simulink model "model"  (R2014a)
(part 2 of 2)

  bus129 : powerlib/Measurements/Load Flow Bus  LConnTagsString=a  ID=bus129  Vbase=110000  Vref=1  Vangle=0  VLF=1  angleLF=0
      settings: AttributesFormatString=|
      | %<ID>
      | %<Vbase>V
      | %<VLF>pu
      | %<angleLF>deg.
      | %<Name>
  bus13 : powerlib/Measurements/Load Flow Bus  LConnTagsString=a  ID=bus13  Vbase=110000  Vref=1  Vangle=0  VLF=1  angleLF=0
      settings: AttributesFormatString=|
      | %<ID>
      | %<Vbase>V
      | %<VLF>pu
      | %<angleLF>deg.
      | %<Name>
  bus130 : powerlib/Measurements/Load Flow Bus  LConnTagsString=a  ID=bus130  Vbase=110000  Vref=1  Vangle=0  VLF=1  angleLF=0
      settings: AttributesFormatString=|
      | %<ID>
      | %<Vbase>V
      | %<VLF>pu
      | %<angleLF>deg.
      | %<Name>
  bus131 : powerlib/Measurements/Load Flow Bus  LConnTagsString=a  ID=bus131  Vbase=110000  Vref=1  Vangle=0  VLF=1  angleLF=0
      settings: AttributesFormatString=|
      | %<ID>
      | %<Vbase>V
      | %<VLF>pu
      | %<angleLF>deg.
      | %<Name>
  bus132 : powerlib/Measurements/Load Flow Bus  LConnTagsString=a  ID=bus132  Vbase=110000  Vref=1  Vangle=0  VLF=1  angleLF=0
      settings: AttributesFormatString=|
      | %<ID>
      | %<Vbase>V
      | %<VLF>pu
      | %<angleLF>deg.
      | %<Name>
  bus133 : powerlib/Measurements/Load Flow Bus  LConnTagsString=a  ID=bus133  Vbase=110000  Vref=1  Vangle=0  VLF=1  angleLF=0
      settings: AttributesFormatString=|
      | %<ID>
      | %<Vbase>V
      | %<VLF>pu
      | %<angleLF>deg.
      | %<Name>
  bus134 : powerlib/Measurements/Load Flow Bus  LConnTagsString=a  ID=bus134  Vbase=110000  Vref=1  Vangle=0  VLF=1  angleLF=0
      settings: AttributesFormatString=|
      | %<ID>
      | %<Vbase>V
      | %<VLF>pu
      | %<angleLF>deg.
      | %<Name>
  bus135 : powerlib/Measurements/Load Flow Bus  LConnTagsString=a  ID=bus135  Vbase=110000  Vref=1  Vangle=0  VLF=1  angleLF=0
      settings: AttributesFormatString=|
      | %<ID>
      | %<Vbase>V
      | %<VLF>pu
      | %<angleLF>deg.
      | %<Name>
  bus136 : powerlib/Measurements/Load Flow Bus  LConnTagsString=a  ID=bus136  Vbase=110000  Vref=1  Vangle=0  VLF=1  angleLF=0
      settings: AttributesFormatString=|
      | %<ID>
      | %<Vbase>V
      | %<VLF>pu
      | %<angleLF>deg.
      | %<Name>
  bus137 : powerlib/Measurements/Load Flow Bus  LConnTagsString=a  ID=bus137  Vbase=110000  Vref=1  Vangle=0  VLF=1  angleLF=0
      settings: AttributesFormatString=|
      | %<ID>
      | %<Vbase>V
      | %<VLF>pu
      | %<angleLF>deg.
      | %<Name>
  bus138 : powerlib/Measurements/Load Flow Bus  LConnTagsString=a  ID=bus138  Vbase=110000  Vref=1  Vangle=0  VLF=1  angleLF=0
      settings: AttributesFormatString=|
      | %<ID>
      | %<Vbase>V
      | %<VLF>pu
      | %<angleLF>deg.
      | %<Name>
  bus139 : powerlib/Measurements/Load Flow Bus  LConnTagsString=a  ID=bus139  Vbase=110000  Vref=1  Vangle=0  VLF=1  angleLF=0
      settings: AttributesFormatString=|
      | %<ID>
      | %<Vbase>V
      | %<VLF>pu
      | %<angleLF>deg.
      | %<Name>
  bus14 : powerlib/Measurements/Load Flow Bus  LConnTagsString=a  ID=bus14  Vbase=110000  Vref=1  Vangle=0  VLF=1  angleLF=0
      settings: AttributesFormatString=|
      | %<ID>
      | %<Vbase>V
      | %<VLF>pu
      | %<angleLF>deg.
      | %<Name>
  bus140 : powerlib/Measurements/Load Flow Bus  LConnTagsString=a  ID=bus140  Vbase=110000  Vref=1  Vangle=0  VLF=1  angleLF=0
      settings: AttributesFormatString=|
      | %<ID>
      | %<Vbase>V
      | %<VLF>pu
      | %<angleLF>deg.
      | %<Name>
  bus141 : powerlib/Measurements/Load Flow Bus  LConnTagsString=a  ID=bus141  Vbase=110000  Vref=1  Vangle=0  VLF=1  angleLF=0
      settings: AttributesFormatString=|
      | %<ID>
      | %<Vbase>V
      | %<VLF>pu
      | %<angleLF>deg.
      | %<Name>
  bus142 : powerlib/Measurements/Load Flow Bus  LConnTagsString=a  ID=bus142  Vbase=110000  Vref=1  Vangle=0  VLF=1  angleLF=0
      settings: AttributesFormatString=|
      | %<ID>
      | %<Vbase>V
      | %<VLF>pu
      | %<angleLF>deg.
      | %<Name>
  bus143 : powerlib/Measurements/Load Flow Bus  LConnTagsString=a  ID=bus143  Vbase=110000  Vref=1  Vangle=0  VLF=1  angleLF=0
      settings: AttributesFormatString=|
      | %<ID>
      | %<Vbase>V
      | %<VLF>pu
      | %<angleLF>deg.
      | %<Name>
  bus144 : powerlib/Measurements/Load Flow Bus  LConnTagsString=a  ID=bus144  Vbase=110000  Vref=1  Vangle=0  VLF=1  angleLF=0
      settings: AttributesFormatString=|
      | %<ID>
      | %<Vbase>V
      | %<VLF>pu
      | %<angleLF>deg.
      | %<Name>
  bus145 : powerlib/Measurements/Load Flow Bus  LConnTagsString=a  ID=bus145  Vbase=110000  Vref=1  Vangle=0  VLF=1  angleLF=0
      settings: AttributesFormatString=|
      | %<ID>
      | %<Vbase>V
      | %<VLF>pu
      | %<angleLF>deg.
      | %<Name>
  bus146 : powerlib/Measurements/Load Flow Bus  LConnTagsString=a  ID=bus146  Vbase=110000  Vref=1  Vangle=0  VLF=1  angleLF=0
      settings: AttributesFormatString=|
      | %<ID>
      | %<Vbase>V
      | %<VLF>pu
      | %<angleLF>deg.
      | %<Name>
  bus147 : powerlib/Measurements/Load Flow Bus  LConnTagsString=a  ID=bus147  Vbase=110000  Vref=1  Vangle=0  VLF=1  angleLF=0
      settings: AttributesFormatString=|
      | %<ID>
      | %<Vbase>V
      | %<VLF>pu
      | %<angleLF>deg.
      | %<Name>
  bus148 : powerlib/Measurements/Load Flow Bus  LConnTagsString=a  ID=bus148  Vbase=110000  Vref=1  Vangle=0  VLF=1  angleLF=0
      settings: AttributesFormatString=|
      | %<ID>
      | %<Vbase>V
      | %<VLF>pu
      | %<angleLF>deg.
      | %<Name>
  bus149 : powerlib/Measurements/Load Flow Bus  LConnTagsString=a  ID=bus149  Vbase=110000  Vref=1  Vangle=0  VLF=1  angleLF=0
      settings: AttributesFormatString=|
      | %<ID>
      | %<Vbase>V
      | %<VLF>pu
      | %<angleLF>deg.
      | %<Name>
  bus15 : powerlib/Measurements/Load Flow Bus  LConnTagsString=a  ID=bus15  Vbase=110000  Vref=1  Vangle=0  VLF=1  angleLF=0
      settings: AttributesFormatString=|
      | %<ID>
      | %<Vbase>V
      | %<VLF>pu
      | %<angleLF>deg.
      | %<Name>
  bus150 : powerlib/Measurements/Load Flow Bus  LConnTagsString=a  ID=bus150  Vbase=110000  Vref=1  Vangle=0  VLF=1  angleLF=0
      settings: AttributesFormatString=|
      | %<ID>
      | %<Vbase>V
      | %<VLF>pu
      | %<angleLF>deg.
      | %<Name>
  bus151 : powerlib/Measurements/Load Flow Bus  LConnTagsString=a  ID=bus151  Vbase=110000  Vref=1  Vangle=0  VLF=1  angleLF=0
      settings: AttributesFormatString=|
      | %<ID>
      | %<Vbase>V
      | %<VLF>pu
      | %<angleLF>deg.
      | %<Name>
  bus152 : powerlib/Measurements/Load Flow Bus  LConnTagsString=a  ID=bus152  Vbase=110000  Vref=1  Vangle=0  VLF=1  angleLF=0
      settings: AttributesFormatString=|
      | %<ID>
      | %<Vbase>V
      | %<VLF>pu
      | %<angleLF>deg.
      | %<Name>
  bus153 : powerlib/Measurements/Load Flow Bus  LConnTagsString=a  ID=bus153  Vbase=110000  Vref=1  Vangle=0  VLF=1  angleLF=0
      settings: AttributesFormatString=|
      | %<ID>
      | %<Vbase>V
      | %<VLF>pu
      | %<angleLF>deg.
      | %<Name>
  bus154 : powerlib/Measurements/Load Flow Bus  LConnTagsString=a  ID=bus154  Vbase=110000  Vref=1  Vangle=0  VLF=1  angleLF=0
      settings: AttributesFormatString=|
      | %<ID>
      | %<Vbase>V
      | %<VLF>pu
      | %<angleLF>deg.
      | %<Name>
  bus155 : powerlib/Measurements/Load Flow Bus  LConnTagsString=a  ID=bus155  Vbase=110000  Vref=1  Vangle=0  VLF=1  angleLF=0
      settings: AttributesFormatString=|
      | %<ID>
      | %<Vbase>V
      | %<VLF>pu
      | %<angleLF>deg.
      | %<Name>
  bus156 : powerlib/Measurements/Load Flow Bus  LConnTagsString=a  ID=bus156  Vbase=110000  Vref=1  Vangle=0  VLF=1  angleLF=0
      settings: AttributesFormatString=|
      | %<ID>
      | %<Vbase>V
      | %<VLF>pu
      | %<angleLF>deg.
      | %<Name>
  bus157 : powerlib/Measurements/Load Flow Bus  LConnTagsString=a  ID=bus157  Vbase=110000  Vref=1  Vangle=0  VLF=1  angleLF=0
      settings: AttributesFormatString=|
      | %<ID>
      | %<Vbase>V
      | %<VLF>pu
      | %<angleLF>deg.
      | %<Name>
  bus158 : powerlib/Measurements/Load Flow Bus  LConnTagsString=a  ID=bus158  Vbase=110000  Vref=1  Vangle=0  VLF=1  angleLF=0
      settings: AttributesFormatString=|
      | %<ID>
      | %<Vbase>V
      | %<VLF>pu
      | %<angleLF>deg.
      | %<Name>
  bus159 : powerlib/Measurements/Load Flow Bus  LConnTagsString=a  ID=bus159  Vbase=110000  Vref=1  Vangle=0  VLF=1  angleLF=0
      settings: AttributesFormatString=|
      | %<ID>
      | %<Vbase>V
      | %<VLF>pu
      | %<angleLF>deg.
      | %<Name>
  bus16 : powerlib/Measurements/Load Flow Bus  LConnTagsString=a  ID=bus16  Vbase=110000  Vref=1  Vangle=0  VLF=1  angleLF=0
      settings: AttributesFormatString=|
      | %<ID>
      | %<Vbase>V
      | %<VLF>pu
      | %<angleLF>deg.
      | %<Name>
  bus160 : powerlib/Measurements/Load Flow Bus  LConnTagsString=a  ID=bus160  Vbase=110000  Vref=1  Vangle=0  VLF=1  angleLF=0
      settings: AttributesFormatString=|
      | %<ID>
      | %<Vbase>V
      | %<VLF>pu
      | %<angleLF>deg.
      | %<Name>
  bus161 : powerlib/Measurements/Load Flow Bus  LConnTagsString=a  ID=bus161  Vbase=110000  Vref=1  Vangle=0  VLF=1  angleLF=0
      settings: AttributesFormatString=|
      | %<ID>
      | %<Vbase>V
      | %<VLF>pu
      | %<angleLF>deg.
      | %<Name>
  bus162 : powerlib/Measurements/Load Flow Bus  LConnTagsString=a  ID=bus162  Vbase=110000  Vref=1  Vangle=0  VLF=1  angleLF=0
      settings: AttributesFormatString=|
      | %<ID>
      | %<Vbase>V
      | %<VLF>pu
      | %<angleLF>deg.
      | %<Name>
  bus163 : powerlib/Measurements/Load Flow Bus  LConnTagsString=a  ID=bus163  Vbase=110000  Vref=1  Vangle=0  VLF=1  angleLF=0
      settings: AttributesFormatString=|
      | %<ID>
      | %<Vbase>V
      | %<VLF>pu
      | %<angleLF>deg.
      | %<Name>
  bus164 : powerlib/Measurements/Load Flow Bus  LConnTagsString=a  ID=bus164  Vbase=110000  Vref=1  Vangle=0  VLF=1  angleLF=0
      settings: AttributesFormatString=|
      | %<ID>
      | %<Vbase>V
      | %<VLF>pu
      | %<angleLF>deg.
      | %<Name>
  bus165 : powerlib/Measurements/Load Flow Bus  LConnTagsString=a  ID=bus165  Vbase=110000  Vref=1  Vangle=0  VLF=1  angleLF=0
      settings: AttributesFormatString=|
      | %<ID>
      | %<Vbase>V
      | %<VLF>pu
      | %<angleLF>deg.
      | %<Name>
  bus166 : powerlib/Measurements/Load Flow Bus  LConnTagsString=a  ID=bus166  Vbase=110000  Vref=1  Vangle=0  VLF=1  angleLF=0
      settings: AttributesFormatString=|
      | %<ID>
      | %<Vbase>V
      | %<VLF>pu
      | %<angleLF>deg.
      | %<Name>
  bus167 : powerlib/Measurements/Load Flow Bus  LConnTagsString=a  ID=bus167  Vbase=110000  Vref=1  Vangle=0  VLF=1  angleLF=0
      settings: AttributesFormatString=|
      | %<ID>
      | %<Vbase>V
      | %<VLF>pu
      | %<angleLF>deg.
      | %<Name>
  bus168 : powerlib/Measurements/Load Flow Bus  LConnTagsString=a  ID=bus168  Vbase=110000  Vref=1  Vangle=0  VLF=1  angleLF=0
      settings: AttributesFormatString=|
      | %<ID>
      | %<Vbase>V
      | %<VLF>pu
      | %<angleLF>deg.
      | %<Name>
  bus169 : powerlib/Measurements/Load Flow Bus  LConnTagsString=a  ID=bus169  Vbase=110000  Vref=1  Vangle=0  VLF=1  angleLF=0
      settings: AttributesFormatString=|
      | %<ID>
      | %<Vbase>V
      | %<VLF>pu
      | %<angleLF>deg.
      | %<Name>
  bus17 : powerlib/Measurements/Load Flow Bus  LConnTagsString=a  ID=bus17  Vbase=110000  Vref=1  Vangle=0  VLF=1  angleLF=0
      settings: AttributesFormatString=|
      | %<ID>
      | %<Vbase>V
      | %<VLF>pu
      | %<angleLF>deg.
      | %<Name>
  bus170 : powerlib/Measurements/Load Flow Bus  LConnTagsString=a  ID=bus170  Vbase=110000  Vref=1  Vangle=0  VLF=1  angleLF=0
      settings: AttributesFormatString=|
      | %<ID>
      | %<Vbase>V
      | %<VLF>pu
      | %<angleLF>deg.
      | %<Name>
  bus171 : powerlib/Measurements/Load Flow Bus  LConnTagsString=a  ID=bus171  Vbase=110000  Vref=1  Vangle=0  VLF=1  angleLF=0
      settings: AttributesFormatString=|
      | %<ID>
      | %<Vbase>V
      | %<VLF>pu
      | %<angleLF>deg.
      | %<Name>
  bus172 : powerlib/Measurements/Load Flow Bus  LConnTagsString=a  ID=bus172  Vbase=110000  Vref=1  Vangle=0  VLF=1  angleLF=0
      settings: AttributesFormatString=|
      | %<ID>
      | %<Vbase>V
      | %<VLF>pu
      | %<angleLF>deg.
      | %<Name>
  bus173 : powerlib/Measurements/Load Flow Bus  LConnTagsString=a  ID=bus173  Vbase=110000  Vref=1  Vangle=0  VLF=1  angleLF=0
      settings: AttributesFormatString=|
      | %<ID>
      | %<Vbase>V
      | %<VLF>pu
      | %<angleLF>deg.
      | %<Name>
  bus174 : powerlib/Measurements/Load Flow Bus  LConnTagsString=a  ID=bus174  Vbase=110000  Vref=1  Vangle=0  VLF=1  angleLF=0
      settings: AttributesFormatString=|
      | %<ID>
      | %<Vbase>V
      | %<VLF>pu
      | %<angleLF>deg.
      | %<Name>
  bus175 : powerlib/Measurements/Load Flow Bus  LConnTagsString=a  ID=bus175  Vbase=110000  Vref=1  Vangle=0  VLF=1  angleLF=0
      settings: AttributesFormatString=|
      | %<ID>
      | %<Vbase>V
      | %<VLF>pu
      | %<angleLF>deg.
      | %<Name>
  bus176 : powerlib/Measurements/Load Flow Bus  LConnTagsString=a  ID=bus176  Vbase=110000  Vref=1  Vangle=0  VLF=1  angleLF=0
      settings: AttributesFormatString=|
      | %<ID>
      | %<Vbase>V
      | %<VLF>pu
      | %<angleLF>deg.
      | %<Name>
  bus177 : powerlib/Measurements/Load Flow Bus  LConnTagsString=a  ID=bus177  Vbase=110000  Vref=1  Vangle=0  VLF=1  angleLF=0
      settings: AttributesFormatString=|
      | %<ID>
      | %<Vbase>V
      | %<VLF>pu
      | %<angleLF>deg.
      | %<Name>
  bus178 : powerlib/Measurements/Load Flow Bus  LConnTagsString=a  ID=bus178  Vbase=110000  Vref=1  Vangle=0  VLF=1  angleLF=0
      settings: AttributesFormatString=|
      | %<ID>
      | %<Vbase>V
      | %<VLF>pu
      | %<angleLF>deg.
      | %<Name>
  bus179 : powerlib/Measurements/Load Flow Bus  LConnTagsString=a  ID=bus179  Vbase=110000  Vref=1  Vangle=0  VLF=1  angleLF=0
      settings: AttributesFormatString=|
      | %<ID>
      | %<Vbase>V
      | %<VLF>pu
      | %<angleLF>deg.
      | %<Name>
  bus18 : powerlib/Measurements/Load Flow Bus  LConnTagsString=a  ID=bus18  Vbase=110000  Vref=1  Vangle=0  VLF=1  angleLF=0
      settings: AttributesFormatString=|
      | %<ID>
      | %<Vbase>V
      | %<VLF>pu
      | %<angleLF>deg.
      | %<Name>
  bus180 : powerlib/Measurements/Load Flow Bus  LConnTagsString=a  ID=bus180  Vbase=110000  Vref=1  Vangle=0  VLF=1  angleLF=0
      settings: AttributesFormatString=|
      | %<ID>
      | %<Vbase>V
      | %<VLF>pu
      | %<angleLF>deg.
      | %<Name>
  bus181 : powerlib/Measurements/Load Flow Bus  LConnTagsString=a  ID=bus181  Vbase=110000  Vref=1  Vangle=0  VLF=1  angleLF=0
      settings: AttributesFormatString=|
      | %<ID>
      | %<Vbase>V
      | %<VLF>pu
      | %<angleLF>deg.
      | %<Name>
  bus182 : powerlib/Measurements/Load Flow Bus  LConnTagsString=a  ID=bus182  Vbase=110000  Vref=1  Vangle=0  VLF=1  angleLF=0
      settings: AttributesFormatString=|
      | %<ID>
      | %<Vbase>V
      | %<VLF>pu
      | %<angleLF>deg.
      | %<Name>
  bus183 : powerlib/Measurements/Load Flow Bus  LConnTagsString=a  ID=bus183  Vbase=110000  Vref=1  Vangle=0  VLF=1  angleLF=0
      settings: AttributesFormatString=|
      | %<ID>
      | %<Vbase>V
      | %<VLF>pu
      | %<angleLF>deg.
      | %<Name>
  bus184 : powerlib/Measurements/Load Flow Bus  LConnTagsString=a  ID=bus184  Vbase=110000  Vref=1  Vangle=0  VLF=1  angleLF=0
      settings: AttributesFormatString=|
      | %<ID>
      | %<Vbase>V
      | %<VLF>pu
      | %<angleLF>deg.
      | %<Name>
  bus185 : powerlib/Measurements/Load Flow Bus  LConnTagsString=a  ID=bus185  Vbase=110000  Vref=1  Vangle=0  VLF=1  angleLF=0
      settings: AttributesFormatString=|
      | %<ID>
      | %<Vbase>V
      | %<VLF>pu
      | %<angleLF>deg.
      | %<Name>
  bus186 : powerlib/Measurements/Load Flow Bus  LConnTagsString=a  ID=bus186  Vbase=110000  Vref=1  Vangle=0  VLF=1  angleLF=0
      settings: AttributesFormatString=|
      | %<ID>
      | %<Vbase>V
      | %<VLF>pu
      | %<angleLF>deg.
      | %<Name>
  bus187 : powerlib/Measurements/Load Flow Bus  LConnTagsString=a  ID=bus187  Vbase=110000  Vref=1  Vangle=0  VLF=1  angleLF=0
      settings: AttributesFormatString=|
      | %<ID>
      | %<Vbase>V
      | %<VLF>pu
      | %<angleLF>deg.
      | %<Name>
  bus188 : powerlib/Measurements/Load Flow Bus  LConnTagsString=a  ID=bus188  Vbase=110000  Vref=1  Vangle=0  VLF=1  angleLF=0
      settings: AttributesFormatString=|
      | %<ID>
      | %<Vbase>V
      | %<VLF>pu
      | %<angleLF>deg.
      | %<Name>
  bus189 : powerlib/Measurements/Load Flow Bus  LConnTagsString=a  ID=bus189  Vbase=110000  Vref=1  Vangle=0  VLF=1  angleLF=0
      settings: AttributesFormatString=|
      | %<ID>
      | %<Vbase>V
      | %<VLF>pu
      | %<angleLF>deg.
      | %<Name>
  bus19 : powerlib/Measurements/Load Flow Bus  LConnTagsString=a  ID=bus19  Vbase=110000  Vref=1  Vangle=0  VLF=1  angleLF=0
      settings: AttributesFormatString=|
      | %<ID>
      | %<Vbase>V
      | %<VLF>pu
      | %<angleLF>deg.
      | %<Name>
  bus190 : powerlib/Measurements/Load Flow Bus  LConnTagsString=a  ID=bus190  Vbase=110000  Vref=1  Vangle=0  VLF=1  angleLF=0
      settings: AttributesFormatString=|
      | %<ID>
      | %<Vbase>V
      | %<VLF>pu
      | %<angleLF>deg.
      | %<Name>
  bus191 : powerlib/Measurements/Load Flow Bus  LConnTagsString=a  ID=bus191  Vbase=220000  Vref=1  Vangle=0  VLF=1  angleLF=0
      settings: AttributesFormatString=|
      | %<ID>
      | %<Vbase>V
      | %<VLF>pu
      | %<angleLF>deg.
      | %<Name>
  bus192 : powerlib/Measurements/Load Flow Bus  LConnTagsString=a  ID=bus192  Vbase=220000  Vref=1  Vangle=0  VLF=1  angleLF=0
      settings: AttributesFormatString=|
      | %<ID>
      | %<Vbase>V
      | %<VLF>pu
      | %<angleLF>deg.
      | %<Name>
  bus193 : powerlib/Measurements/Load Flow Bus  LConnTagsString=a  ID=bus193  Vbase=220000  Vref=1  Vangle=0  VLF=1  angleLF=0
      settings: AttributesFormatString=|
      | %<ID>
      | %<Vbase>V
      | %<VLF>pu
      | %<angleLF>deg.
      | %<Name>
  bus194 : powerlib/Measurements/Load Flow Bus  LConnTagsString=a  ID=bus194  Vbase=220000  Vref=1  Vangle=0  VLF=1  angleLF=0
      settings: AttributesFormatString=|
      | %<ID>
      | %<Vbase>V
      | %<VLF>pu
      | %<angleLF>deg.
      | %<Name>
  bus195 : powerlib/Measurements/Load Flow Bus  LConnTagsString=a  ID=bus195  Vbase=220000  Vref=1  Vangle=0  VLF=1  angleLF=0
      settings: AttributesFormatString=|
      | %<ID>
      | %<Vbase>V
      | %<VLF>pu
      | %<angleLF>deg.
      | %<Name>
  bus196 : powerlib/Measurements/Load Flow Bus  LConnTagsString=a  ID=bus196  Vbase=220000  Vref=1  Vangle=0  VLF=1  angleLF=0
      settings: AttributesFormatString=|
      | %<ID>
      | %<Vbase>V
      | %<VLF>pu
      | %<angleLF>deg.
      | %<Name>
  bus197 : powerlib/Measurements/Load Flow Bus  LConnTagsString=a  ID=bus197  Vbase=220000  Vref=1  Vangle=0  VLF=1  angleLF=0
      settings: AttributesFormatString=|
      | %<ID>
      | %<Vbase>V
      | %<VLF>pu
      | %<angleLF>deg.
      | %<Name>
  bus198 : powerlib/Measurements/Load Flow Bus  LConnTagsString=a  ID=bus198  Vbase=220000  Vref=1  Vangle=0  VLF=1  angleLF=0
      settings: AttributesFormatString=|
      | %<ID>
      | %<Vbase>V
      | %<VLF>pu
      | %<angleLF>deg.
      | %<Name>
  bus199 : powerlib/Measurements/Load Flow Bus  LConnTagsString=a  ID=bus199  Vbase=220000  Vref=1  Vangle=0  VLF=1  angleLF=0
      settings: AttributesFormatString=|
      | %<ID>
      | %<Vbase>V
      | %<VLF>pu
      | %<angleLF>deg.
      | %<Name>
  bus2 : powerlib/Measurements/Load Flow Bus  LConnTagsString=a  ID=bus2  Vbase=110000  Vref=1  Vangle=0  VLF=1  angleLF=0
      settings: AttributesFormatString=|
      | %<ID>
      | %<Vbase>V
      | %<VLF>pu
      | %<angleLF>deg.
      | %<Name>
  bus20 : powerlib/Measurements/Load Flow Bus  LConnTagsString=a  ID=bus20  Vbase=110000  Vref=1  Vangle=0  VLF=1  angleLF=0
      settings: AttributesFormatString=|
      | %<ID>
      | %<Vbase>V
      | %<VLF>pu
      | %<angleLF>deg.
      | %<Name>
  bus200 : powerlib/Measurements/Load Flow Bus  LConnTagsString=a  ID=bus200  Vbase=220000  Vref=1  Vangle=0  VLF=1  angleLF=0
      settings: AttributesFormatString=|
      | %<ID>
      | %<Vbase>V
      | %<VLF>pu
      | %<angleLF>deg.
      | %<Name>
  bus201 : powerlib/Measurements/Load Flow Bus  LConnTagsString=a  ID=bus201  Vbase=220000  Vref=1  Vangle=0  VLF=1  angleLF=0
      settings: AttributesFormatString=|
      | %<ID>
      | %<Vbase>V
      | %<VLF>pu
      | %<angleLF>deg.
      | %<Name>
  bus202 : powerlib/Measurements/Load Flow Bus  LConnTagsString=a  ID=bus202  Vbase=220000  Vref=1  Vangle=0  VLF=1  angleLF=0
      settings: AttributesFormatString=|
      | %<ID>
      | %<Vbase>V
      | %<VLF>pu
      | %<angleLF>deg.
      | %<Name>
  bus203 : powerlib/Measurements/Load Flow Bus  LConnTagsString=a  ID=bus203  Vbase=220000  Vref=1  Vangle=0  VLF=1  angleLF=0
      settings: AttributesFormatString=|
      | %<ID>
      | %<Vbase>V
      | %<VLF>pu
      | %<angleLF>deg.
      | %<Name>
  bus204 : powerlib/Measurements/Load Flow Bus  LConnTagsString=a  ID=bus204  Vbase=220000  Vref=1  Vangle=0  VLF=1  angleLF=0
      settings: AttributesFormatString=|
      | %<ID>
      | %<Vbase>V
      | %<VLF>pu
      | %<angleLF>deg.
      | %<Name>
  bus205 : powerlib/Measurements/Load Flow Bus  LConnTagsString=a  ID=bus205  Vbase=220000  Vref=1  Vangle=0  VLF=1  angleLF=0
      settings: AttributesFormatString=|
      | %<ID>
      | %<Vbase>V
      | %<VLF>pu
      | %<angleLF>deg.
      | %<Name>
  bus206 : powerlib/Measurements/Load Flow Bus  LConnTagsString=a  ID=bus206  Vbase=220000  Vref=1  Vangle=0  VLF=1  angleLF=0
      settings: AttributesFormatString=|
      | %<ID>
      | %<Vbase>V
      | %<VLF>pu
      | %<angleLF>deg.
      | %<Name>
  bus207 : powerlib/Measurements/Load Flow Bus  LConnTagsString=a  ID=bus207  Vbase=220000  Vref=1  Vangle=0  VLF=1  angleLF=0
      settings: AttributesFormatString=|
      | %<ID>
      | %<Vbase>V
      | %<VLF>pu
      | %<angleLF>deg.
      | %<Name>
  bus208 : powerlib/Measurements/Load Flow Bus  LConnTagsString=a  ID=bus208  Vbase=220000  Vref=1  Vangle=0  VLF=1  angleLF=0
      settings: AttributesFormatString=|
      | %<ID>
      | %<Vbase>V
      | %<VLF>pu
      | %<angleLF>deg.
      | %<Name>
  bus209 : powerlib/Measurements/Load Flow Bus  LConnTagsString=a  ID=bus209  Vbase=220000  Vref=1  Vangle=0  VLF=1  angleLF=0
      settings: AttributesFormatString=|
      | %<ID>
      | %<Vbase>V
      | %<VLF>pu
      | %<angleLF>deg.
      | %<Name>
  bus21 : powerlib/Measurements/Load Flow Bus  LConnTagsString=a  ID=bus21  Vbase=110000  Vref=1  Vangle=0  VLF=1  angleLF=0
      settings: AttributesFormatString=|
      | %<ID>
      | %<Vbase>V
      | %<VLF>pu
      | %<angleLF>deg.
      | %<Name>
  bus210 : powerlib/Measurements/Load Flow Bus  LConnTagsString=a  ID=bus210  Vbase=220000  Vref=1  Vangle=0  VLF=1  angleLF=0
      settings: AttributesFormatString=|
      | %<ID>
      | %<Vbase>V
      | %<VLF>pu
      | %<angleLF>deg.
      | %<Name>
  bus211 : powerlib/Measurements/Load Flow Bus  LConnTagsString=a  ID=bus211  Vbase=220000  Vref=1  Vangle=0  VLF=1  angleLF=0
      settings: AttributesFormatString=|
      | %<ID>
      | %<Vbase>V
      | %<VLF>pu
      | %<angleLF>deg.
      | %<Name>
  bus212 : powerlib/Measurements/Load Flow Bus  LConnTagsString=a  ID=bus212  Vbase=220000  Vref=1  Vangle=0  VLF=1  angleLF=0
      settings: AttributesFormatString=|
      | %<ID>
      | %<Vbase>V
      | %<VLF>pu
      | %<angleLF>deg.
      | %<Name>
  bus213 : powerlib/Measurements/Load Flow Bus  LConnTagsString=a  ID=bus213  Vbase=220000  Vref=1  Vangle=0  VLF=1  angleLF=0
      settings: AttributesFormatString=|
      | %<ID>
      | %<Vbase>V
      | %<VLF>pu
      | %<angleLF>deg.
      | %<Name>
  bus214 : powerlib/Measurements/Load Flow Bus  LConnTagsString=a  ID=bus214  Vbase=220000  Vref=1  Vangle=0  VLF=1  angleLF=0
      settings: AttributesFormatString=|
      | %<ID>
      | %<Vbase>V
      | %<VLF>pu
      | %<angleLF>deg.
      | %<Name>
  bus215 : powerlib/Measurements/Load Flow Bus  LConnTagsString=a  ID=bus215  Vbase=220000  Vref=1  Vangle=0  VLF=1  angleLF=0
      settings: AttributesFormatString=|
      | %<ID>
      | %<Vbase>V
      | %<VLF>pu
      | %<angleLF>deg.
      | %<Name>
  bus216 : powerlib/Measurements/Load Flow Bus  LConnTagsString=a  ID=bus216  Vbase=220000  Vref=1  Vangle=0  VLF=1  angleLF=0
      settings: AttributesFormatString=|
      | %<ID>
      | %<Vbase>V
      | %<VLF>pu
      | %<angleLF>deg.
      | %<Name>
  bus217 : powerlib/Measurements/Load Flow Bus  LConnTagsString=a  ID=bus217  Vbase=220000  Vref=1  Vangle=0  VLF=1  angleLF=0
      settings: AttributesFormatString=|
      | %<ID>
      | %<Vbase>V
      | %<VLF>pu
      | %<angleLF>deg.
      | %<Name>
  bus218 : powerlib/Measurements/Load Flow Bus  LConnTagsString=a  ID=bus218  Vbase=220000  Vref=1  Vangle=0  VLF=1  angleLF=0
      settings: AttributesFormatString=|
      | %<ID>
      | %<Vbase>V
      | %<VLF>pu
      | %<angleLF>deg.
      | %<Name>
  bus219 : powerlib/Measurements/Load Flow Bus  LConnTagsString=a  ID=bus219  Vbase=220000  Vref=1  Vangle=0  VLF=1  angleLF=0
      settings: AttributesFormatString=|
      | %<ID>
      | %<Vbase>V
      | %<VLF>pu
      | %<angleLF>deg.
      | %<Name>
  bus22 : powerlib/Measurements/Load Flow Bus  LConnTagsString=a  ID=bus22  Vbase=110000  Vref=1  Vangle=0  VLF=1  angleLF=0
      settings: AttributesFormatString=|
      | %<ID>
      | %<Vbase>V
      | %<VLF>pu
      | %<angleLF>deg.
      | %<Name>
  bus220 : powerlib/Measurements/Load Flow Bus  LConnTagsString=a  ID=bus220  Vbase=220000  Vref=1  Vangle=0  VLF=1  angleLF=0
      settings: AttributesFormatString=|
      | %<ID>
      | %<Vbase>V
      | %<VLF>pu
      | %<angleLF>deg.
      | %<Name>
  bus221 : powerlib/Measurements/Load Flow Bus  LConnTagsString=a  ID=bus221  Vbase=220000  Vref=1  Vangle=0  VLF=1  angleLF=0
      settings: AttributesFormatString=|
      | %<ID>
      | %<Vbase>V
      | %<VLF>pu
      | %<angleLF>deg.
      | %<Name>
  bus222 : powerlib/Measurements/Load Flow Bus  LConnTagsString=a  ID=bus222  Vbase=220000  Vref=1  Vangle=0  VLF=1  angleLF=0
      settings: AttributesFormatString=|
      | %<ID>
      | %<Vbase>V
      | %<VLF>pu
      | %<angleLF>deg.
      | %<Name>
  bus223 : powerlib/Measurements/Load Flow Bus  LConnTagsString=a  ID=bus223  Vbase=220000  Vref=1  Vangle=0  VLF=1  angleLF=0
      settings: AttributesFormatString=|
      | %<ID>
      | %<Vbase>V
      | %<VLF>pu
      | %<angleLF>deg.
      | %<Name>
  bus224 : powerlib/Measurements/Load Flow Bus  LConnTagsString=a  ID=bus224  Vbase=220000  Vref=1  Vangle=0  VLF=1  angleLF=0
      settings: AttributesFormatString=|
      | %<ID>
      | %<Vbase>V
      | %<VLF>pu
      | %<angleLF>deg.
      | %<Name>
  bus225 : powerlib/Measurements/Load Flow Bus  LConnTagsString=a  ID=bus225  Vbase=220000  Vref=1  Vangle=0  VLF=1  angleLF=0
      settings: AttributesFormatString=|
      | %<ID>
      | %<Vbase>V
      | %<VLF>pu
      | %<angleLF>deg.
      | %<Name>
  bus226 : powerlib/Measurements/Load Flow Bus  LConnTagsString=a  ID=bus226  Vbase=220000  Vref=1  Vangle=0  VLF=1  angleLF=0
      settings: AttributesFormatString=|
      | %<ID>
      | %<Vbase>V
      | %<VLF>pu
      | %<angleLF>deg.
      | %<Name>
  bus227 : powerlib/Measurements/Load Flow Bus  LConnTagsString=a  ID=bus227  Vbase=220000  Vref=1  Vangle=0  VLF=1  angleLF=0
      settings: AttributesFormatString=|
      | %<ID>
      | %<Vbase>V
      | %<VLF>pu
      | %<angleLF>deg.
      | %<Name>
  bus23 : powerlib/Measurements/Load Flow Bus  LConnTagsString=a  ID=bus23  Vbase=110000  Vref=1  Vangle=0  VLF=1  angleLF=0
      settings: AttributesFormatString=|
      | %<ID>
      | %<Vbase>V
      | %<VLF>pu
      | %<angleLF>deg.
      | %<Name>
  bus24 : powerlib/Measurements/Load Flow Bus  LConnTagsString=a  ID=bus24  Vbase=110000  Vref=1  Vangle=0  VLF=1  angleLF=0
      settings: AttributesFormatString=|
      | %<ID>
      | %<Vbase>V
      | %<VLF>pu
      | %<angleLF>deg.
      | %<Name>
  bus25 : powerlib/Measurements/Load Flow Bus  LConnTagsString=a  ID=bus25  Vbase=110000  Vref=1  Vangle=0  VLF=1  angleLF=0
      settings: AttributesFormatString=|
      | %<ID>
      | %<Vbase>V
      | %<VLF>pu
      | %<angleLF>deg.
      | %<Name>
  bus26 : powerlib/Measurements/Load Flow Bus  LConnTagsString=a  ID=bus26  Vbase=110000  Vref=1  Vangle=0  VLF=1  angleLF=0
      settings: AttributesFormatString=|
      | %<ID>
      | %<Vbase>V
      | %<VLF>pu
      | %<angleLF>deg.
      | %<Name>
  bus27 : powerlib/Measurements/Load Flow Bus  LConnTagsString=a  ID=bus27  Vbase=110000  Vref=1  Vangle=0  VLF=1  angleLF=0
      settings: AttributesFormatString=|
      | %<ID>
      | %<Vbase>V
      | %<VLF>pu
      | %<angleLF>deg.
      | %<Name>
  bus28 : powerlib/Measurements/Load Flow Bus  LConnTagsString=a  ID=bus28  Vbase=110000  Vref=1  Vangle=0  VLF=1  angleLF=0
      settings: AttributesFormatString=|
      | %<ID>
      | %<Vbase>V
      | %<VLF>pu
      | %<angleLF>deg.
      | %<Name>
  bus29 : powerlib/Measurements/Load Flow Bus  LConnTagsString=a  ID=bus29  Vbase=110000  Vref=1  Vangle=0  VLF=1  angleLF=0
      settings: AttributesFormatString=|
      | %<ID>
      | %<Vbase>V
      | %<VLF>pu
      | %<angleLF>deg.
      | %<Name>
  bus3 : powerlib/Measurements/Load Flow Bus  LConnTagsString=a  ID=bus3  Vbase=110000  Vref=1  Vangle=0  VLF=1  angleLF=0
      settings: AttributesFormatString=|
      | %<ID>
      | %<Vbase>V
      | %<VLF>pu
      | %<angleLF>deg.
      | %<Name>
  bus30 : powerlib/Measurements/Load Flow Bus  LConnTagsString=a  ID=bus30  Vbase=110000  Vref=1  Vangle=0  VLF=1  angleLF=0
      settings: AttributesFormatString=|
      | %<ID>
      | %<Vbase>V
      | %<VLF>pu
      | %<angleLF>deg.
      | %<Name>
  bus31 : powerlib/Measurements/Load Flow Bus  LConnTagsString=a  ID=bus31  Vbase=110000  Vref=1  Vangle=0  VLF=1  angleLF=0
      settings: AttributesFormatString=|
      | %<ID>
      | %<Vbase>V
      | %<VLF>pu
      | %<angleLF>deg.
      | %<Name>
  bus32 : powerlib/Measurements/Load Flow Bus  LConnTagsString=a  ID=bus32  Vbase=110000  Vref=1  Vangle=0  VLF=1  angleLF=0
      settings: AttributesFormatString=|
      | %<ID>
      | %<Vbase>V
      | %<VLF>pu
      | %<angleLF>deg.
      | %<Name>
  bus33 : powerlib/Measurements/Load Flow Bus  LConnTagsString=a  ID=bus33  Vbase=110000  Vref=1  Vangle=0  VLF=1  angleLF=0
      settings: AttributesFormatString=|
      | %<ID>
      | %<Vbase>V
      | %<VLF>pu
      | %<angleLF>deg.
      | %<Name>
  bus34 : powerlib/Measurements/Load Flow Bus  LConnTagsString=a  ID=bus34  Vbase=110000  Vref=1  Vangle=0  VLF=1  angleLF=0
      settings: AttributesFormatString=|
      | %<ID>
      | %<Vbase>V
      | %<VLF>pu
      | %<angleLF>deg.
      | %<Name>
  bus35 : powerlib/Measurements/Load Flow Bus  LConnTagsString=a  ID=bus35  Vbase=110000  Vref=1  Vangle=0  VLF=1  angleLF=0
      settings: AttributesFormatString=|
      | %<ID>
      | %<Vbase>V
      | %<VLF>pu
      | %<angleLF>deg.
      | %<Name>
  bus36 : powerlib/Measurements/Load Flow Bus  LConnTagsString=a  ID=bus36  Vbase=110000  Vref=1  Vangle=0  VLF=1  angleLF=0
      settings: AttributesFormatString=|
      | %<ID>
      | %<Vbase>V
      | %<VLF>pu
      | %<angleLF>deg.
      | %<Name>
  bus37 : powerlib/Measurements/Load Flow Bus  LConnTagsString=a  ID=bus37  Vbase=110000  Vref=1  Vangle=0  VLF=1  angleLF=0
      settings: AttributesFormatString=|
      | %<ID>
      | %<Vbase>V
      | %<VLF>pu
      | %<angleLF>deg.
      | %<Name>
  bus38 : powerlib/Measurements/Load Flow Bus  LConnTagsString=a  ID=bus38  Vbase=110000  Vref=1  Vangle=0  VLF=1  angleLF=0
      settings: AttributesFormatString=|
      | %<ID>
      | %<Vbase>V
      | %<VLF>pu
      | %<angleLF>deg.
      | %<Name>
  bus39 : powerlib/Measurements/Load Flow Bus  LConnTagsString=a  ID=bus39  Vbase=110000  Vref=1  Vangle=0  VLF=1  angleLF=0
      settings: AttributesFormatString=|
      | %<ID>
      | %<Vbase>V
      | %<VLF>pu
      | %<angleLF>deg.
      | %<Name>
  bus4 : powerlib/Measurements/Load Flow Bus  LConnTagsString=a  ID=bus4  Vbase=110000  Vref=1  Vangle=0  VLF=1  angleLF=0
      settings: AttributesFormatString=|
      | %<ID>
      | %<Vbase>V
      | %<VLF>pu
      | %<angleLF>deg.
      | %<Name>
  bus40 : powerlib/Measurements/Load Flow Bus  LConnTagsString=a  ID=bus40  Vbase=110000  Vref=1  Vangle=0  VLF=1  angleLF=0
      settings: AttributesFormatString=|
      | %<ID>
      | %<Vbase>V
      | %<VLF>pu
      | %<angleLF>deg.
      | %<Name>
  bus41 : powerlib/Measurements/Load Flow Bus  LConnTagsString=a  ID=bus41  Vbase=110000  Vref=1  Vangle=0  VLF=1  angleLF=0
      settings: AttributesFormatString=|
      | %<ID>
      | %<Vbase>V
      | %<VLF>pu
      | %<angleLF>deg.
      | %<Name>
  bus42 : powerlib/Measurements/Load Flow Bus  LConnTagsString=a  ID=bus42  Vbase=110000  Vref=1  Vangle=0  VLF=1  angleLF=0
      settings: AttributesFormatString=|
      | %<ID>
      | %<Vbase>V
      | %<VLF>pu
      | %<angleLF>deg.
      | %<Name>
  bus43 : powerlib/Measurements/Load Flow Bus  LConnTagsString=a  ID=bus43  Vbase=110000  Vref=1  Vangle=0  VLF=1  angleLF=0
      settings: AttributesFormatString=|
      | %<ID>
      | %<Vbase>V
      | %<VLF>pu
      | %<angleLF>deg.
      | %<Name>
  bus44 : powerlib/Measurements/Load Flow Bus  LConnTagsString=a  ID=bus44  Vbase=110000  Vref=1  Vangle=0  VLF=1  angleLF=0
      settings: AttributesFormatString=|
      | %<ID>
      | %<Vbase>V
      | %<VLF>pu
      | %<angleLF>deg.
      | %<Name>
  bus45 : powerlib/Measurements/Load Flow Bus  LConnTagsString=a  ID=bus45  Vbase=110000  Vref=1  Vangle=0  VLF=1  angleLF=0
      settings: AttributesFormatString=|
      | %<ID>
      | %<Vbase>V
      | %<VLF>pu
      | %<angleLF>deg.
      | %<Name>
  bus46 : powerlib/Measurements/Load Flow Bus  LConnTagsString=a  ID=bus46  Vbase=110000  Vref=1  Vangle=0  VLF=1  angleLF=0
      settings: AttributesFormatString=|
      | %<ID>
      | %<Vbase>V
      | %<VLF>pu
      | %<angleLF>deg.
      | %<Name>
  bus47 : powerlib/Measurements/Load Flow Bus  LConnTagsString=a  ID=bus47  Vbase=110000  Vref=1  Vangle=0  VLF=1  angleLF=0
      settings: AttributesFormatString=|
      | %<ID>
      | %<Vbase>V
      | %<VLF>pu
      | %<angleLF>deg.
      | %<Name>
  bus48 : powerlib/Measurements/Load Flow Bus  LConnTagsString=a  ID=bus48  Vbase=110000  Vref=1  Vangle=0  VLF=1  angleLF=0
      settings: AttributesFormatString=|
      | %<ID>
      | %<Vbase>V
      | %<VLF>pu
      | %<angleLF>deg.
      | %<Name>
  bus49 : powerlib/Measurements/Load Flow Bus  LConnTagsString=a  ID=bus49  Vbase=110000  Vref=1  Vangle=0  VLF=1  angleLF=0
      settings: AttributesFormatString=|
      | %<ID>
      | %<Vbase>V
      | %<VLF>pu
      | %<angleLF>deg.
      | %<Name>
  bus5 : powerlib/Measurements/Load Flow Bus  LConnTagsString=a  ID=bus5  Vbase=110000  Vref=1  Vangle=0  VLF=1  angleLF=0
      settings: AttributesFormatString=|
      | %<ID>
      | %<Vbase>V
      | %<VLF>pu
      | %<angleLF>deg.
      | %<Name>
  bus50 : powerlib/Measurements/Load Flow Bus  LConnTagsString=a  ID=bus50  Vbase=110000  Vref=1  Vangle=0  VLF=1  angleLF=0
      settings: AttributesFormatString=|
      | %<ID>
      | %<Vbase>V
      | %<VLF>pu
      | %<angleLF>deg.
      | %<Name>
  bus51 : powerlib/Measurements/Load Flow Bus  LConnTagsString=a  ID=bus51  Vbase=110000  Vref=1  Vangle=0  VLF=1  angleLF=0
      settings: AttributesFormatString=|
      | %<ID>
      | %<Vbase>V
      | %<VLF>pu
      | %<angleLF>deg.
      | %<Name>
  bus52 : powerlib/Measurements/Load Flow Bus  LConnTagsString=a  ID=bus52  Vbase=110000  Vref=1  Vangle=0  VLF=1  angleLF=0
      settings: AttributesFormatString=|
      | %<ID>
      | %<Vbase>V
      | %<VLF>pu
      | %<angleLF>deg.
      | %<Name>
  bus53 : powerlib/Measurements/Load Flow Bus  LConnTagsString=a  ID=bus53  Vbase=110000  Vref=1  Vangle=0  VLF=1  angleLF=0
      settings: AttributesFormatString=|
      | %<ID>
      | %<Vbase>V
      | %<VLF>pu
      | %<angleLF>deg.
      | %<Name>
  bus54 : powerlib/Measurements/Load Flow Bus  LConnTagsString=a  ID=bus54  Vbase=110000  Vref=1  Vangle=0  VLF=1  angleLF=0
      settings: AttributesFormatString=|
      | %<ID>
      | %<Vbase>V
      | %<VLF>pu
      | %<angleLF>deg.
      | %<Name>
  bus55 : powerlib/Measurements/Load Flow Bus  LConnTagsString=a  ID=bus55  Vbase=110000  Vref=1  Vangle=0  VLF=1  angleLF=0
      settings: AttributesFormatString=|
      | %<ID>
      | %<Vbase>V
      | %<VLF>pu
      | %<angleLF>deg.
      | %<Name>
  bus56 : powerlib/Measurements/Load Flow Bus  LConnTagsString=a  ID=bus56  Vbase=110000  Vref=1  Vangle=0  VLF=1  angleLF=0
      settings: AttributesFormatString=|
      | %<ID>
      | %<Vbase>V
      | %<VLF>pu
      | %<angleLF>deg.
      | %<Name>
  bus57 : powerlib/Measurements/Load Flow Bus  LConnTagsString=a  ID=bus57  Vbase=110000  Vref=1  Vangle=0  VLF=1  angleLF=0
      settings: AttributesFormatString=|
      | %<ID>
      | %<Vbase>V
      | %<VLF>pu
      | %<angleLF>deg.
      | %<Name>
  bus58 : powerlib/Measurements/Load Flow Bus  LConnTagsString=a  ID=bus58  Vbase=110000  Vref=1  Vangle=0  VLF=1  angleLF=0
      settings: AttributesFormatString=|
      | %<ID>
      | %<Vbase>V
      | %<VLF>pu
      | %<angleLF>deg.
      | %<Name>
  bus59 : powerlib/Measurements/Load Flow Bus  LConnTagsString=a  ID=bus59  Vbase=110000  Vref=1  Vangle=0  VLF=1  angleLF=0
      settings: AttributesFormatString=|
      | %<ID>
      | %<Vbase>V
      | %<VLF>pu
      | %<angleLF>deg.
      | %<Name>
  bus6 : powerlib/Measurements/Load Flow Bus  LConnTagsString=a  ID=bus6  Vbase=110000  Vref=1  Vangle=0  VLF=1  angleLF=0
      settings: AttributesFormatString=|
      | %<ID>
      | %<Vbase>V
      | %<VLF>pu
      | %<angleLF>deg.
      | %<Name>
  bus60 : powerlib/Measurements/Load Flow Bus  LConnTagsString=a  ID=bus60  Vbase=110000  Vref=1  Vangle=0  VLF=1  angleLF=0
      settings: AttributesFormatString=|
      | %<ID>
      | %<Vbase>V
      | %<VLF>pu
      | %<angleLF>deg.
      | %<Name>
  bus61 : powerlib/Measurements/Load Flow Bus  LConnTagsString=a  ID=bus61  Vbase=110000  Vref=1  Vangle=0  VLF=1  angleLF=0
      settings: AttributesFormatString=|
      | %<ID>
      | %<Vbase>V
      | %<VLF>pu
      | %<angleLF>deg.
      | %<Name>
  bus62 : powerlib/Measurements/Load Flow Bus  LConnTagsString=a  ID=bus62  Vbase=110000  Vref=1  Vangle=0  VLF=1  angleLF=0
      settings: AttributesFormatString=|
      | %<ID>
      | %<Vbase>V
      | %<VLF>pu
      | %<angleLF>deg.
      | %<Name>
  bus63 : powerlib/Measurements/Load Flow Bus  LConnTagsString=a  ID=bus63  Vbase=110000  Vref=1  Vangle=0  VLF=1  angleLF=0
      settings: AttributesFormatString=|
      | %<ID>
      | %<Vbase>V
      | %<VLF>pu
      | %<angleLF>deg.
      | %<Name>
  bus64 : powerlib/Measurements/Load Flow Bus  LConnTagsString=a  ID=bus64  Vbase=110000  Vref=1  Vangle=0  VLF=1  angleLF=0
      settings: AttributesFormatString=|
      | %<ID>
      | %<Vbase>V
      | %<VLF>pu
      | %<angleLF>deg.
      | %<Name>
  bus65 : powerlib/Measurements/Load Flow Bus  LConnTagsString=a  ID=bus65  Vbase=110000  Vref=1  Vangle=0  VLF=1  angleLF=0
      settings: AttributesFormatString=|
      | %<ID>
      | %<Vbase>V
      | %<VLF>pu
      | %<angleLF>deg.
      | %<Name>
  bus66 : powerlib/Measurements/Load Flow Bus  LConnTagsString=a  ID=bus66  Vbase=110000  Vref=1  Vangle=0  VLF=1  angleLF=0
      settings: AttributesFormatString=|
      | %<ID>
      | %<Vbase>V
      | %<VLF>pu
      | %<angleLF>deg.
      | %<Name>
  bus67 : powerlib/Measurements/Load Flow Bus  LConnTagsString=a  ID=bus67  Vbase=110000  Vref=1  Vangle=0  VLF=1  angleLF=0
      settings: AttributesFormatString=|
      | %<ID>
      | %<Vbase>V
      | %<VLF>pu
      | %<angleLF>deg.
      | %<Name>
  bus68 : powerlib/Measurements/Load Flow Bus  LConnTagsString=a  ID=bus68  Vbase=110000  Vref=1  Vangle=0  VLF=1  angleLF=0
      settings: AttributesFormatString=|
      | %<ID>
      | %<Vbase>V
      | %<VLF>pu
      | %<angleLF>deg.
      | %<Name>
  bus69 : powerlib/Measurements/Load Flow Bus  LConnTagsString=a  ID=bus69  Vbase=110000  Vref=1  Vangle=0  VLF=1  angleLF=0
      settings: AttributesFormatString=|
      | %<ID>
      | %<Vbase>V
      | %<VLF>pu
      | %<angleLF>deg.
      | %<Name>
  bus7 : powerlib/Measurements/Load Flow Bus  LConnTagsString=a  ID=bus7  Vbase=110000  Vref=1  Vangle=0  VLF=1  angleLF=0
      settings: AttributesFormatString=|
      | %<ID>
      | %<Vbase>V
      | %<VLF>pu
      | %<angleLF>deg.
      | %<Name>
  bus70 : powerlib/Measurements/Load Flow Bus  LConnTagsString=a  ID=bus70  Vbase=110000  Vref=1  Vangle=0  VLF=1  angleLF=0
      settings: AttributesFormatString=|
      | %<ID>
      | %<Vbase>V
      | %<VLF>pu
      | %<angleLF>deg.
      | %<Name>
  bus71 : powerlib/Measurements/Load Flow Bus  LConnTagsString=a  ID=bus71  Vbase=110000  Vref=1  Vangle=0  VLF=1  angleLF=0
      settings: AttributesFormatString=|
      | %<ID>
      | %<Vbase>V
      | %<VLF>pu
      | %<angleLF>deg.
      | %<Name>
  bus72 : powerlib/Measurements/Load Flow Bus  LConnTagsString=a  ID=bus72  Vbase=110000  Vref=1  Vangle=0  VLF=1  angleLF=0
      settings: AttributesFormatString=|
      | %<ID>
      | %<Vbase>V
      | %<VLF>pu
      | %<angleLF>deg.
      | %<Name>
  bus73 : powerlib/Measurements/Load Flow Bus  LConnTagsString=a  ID=bus73  Vbase=110000  Vref=1  Vangle=0  VLF=1  angleLF=0
      settings: AttributesFormatString=|
      | %<ID>
      | %<Vbase>V
      | %<VLF>pu
      | %<angleLF>deg.
      | %<Name>
  bus74 : powerlib/Measurements/Load Flow Bus  LConnTagsString=a  ID=bus74  Vbase=220000  Vref=1  Vangle=0  VLF=1  angleLF=0
      settings: AttributesFormatString=|
      | %<ID>
      | %<Vbase>V
      | %<VLF>pu
      | %<angleLF>deg.
      | %<Name>
  bus75 : powerlib/Measurements/Load Flow Bus  LConnTagsString=a  ID=bus75  Vbase=220000  Vref=1  Vangle=0  VLF=1  angleLF=0
      settings: AttributesFormatString=|
      | %<ID>
      | %<Vbase>V
      | %<VLF>pu
      | %<angleLF>deg.
      | %<Name>
  bus76 : powerlib/Measurements/Load Flow Bus  LConnTagsString=a  ID=bus76  Vbase=220000  Vref=1  Vangle=0  VLF=1  angleLF=0
      settings: AttributesFormatString=|
      | %<ID>
      | %<Vbase>V
      | %<VLF>pu
      | %<angleLF>deg.
      | %<Name>
  bus77 : powerlib/Measurements/Load Flow Bus  LConnTagsString=a  ID=bus77  Vbase=220000  Vref=1  Vangle=0  VLF=1  angleLF=0
      settings: AttributesFormatString=|
      | %<ID>
      | %<Vbase>V
      | %<VLF>pu
      | %<angleLF>deg.
      | %<Name>
  bus78 : powerlib/Measurements/Load Flow Bus  LConnTagsString=a  ID=bus78  Vbase=220000  Vref=1  Vangle=0  VLF=1  angleLF=0
      settings: AttributesFormatString=|
      | %<ID>
      | %<Vbase>V
      | %<VLF>pu
      | %<angleLF>deg.
      | %<Name>
  bus79 : powerlib/Measurements/Load Flow Bus  LConnTagsString=a  ID=bus79  Vbase=220000  Vref=1  Vangle=0  VLF=1  angleLF=0
      settings: AttributesFormatString=|
      | %<ID>
      | %<Vbase>V
      | %<VLF>pu
      | %<angleLF>deg.
      | %<Name>
  bus8 : powerlib/Measurements/Load Flow Bus  LConnTagsString=a  ID=bus8  Vbase=110000  Vref=1  Vangle=0  VLF=1  angleLF=0
      settings: AttributesFormatString=|
      | %<ID>
      | %<Vbase>V
      | %<VLF>pu
      | %<angleLF>deg.
      | %<Name>
  bus80 : powerlib/Measurements/Load Flow Bus  LConnTagsString=a  ID=bus80  Vbase=220000  Vref=1  Vangle=0  VLF=1  angleLF=0
      settings: AttributesFormatString=|
      | %<ID>
      | %<Vbase>V
      | %<VLF>pu
      | %<angleLF>deg.
      | %<Name>
  bus81 : powerlib/Measurements/Load Flow Bus  LConnTagsString=a  ID=bus81  Vbase=220000  Vref=1  Vangle=0  VLF=1  angleLF=0
      settings: AttributesFormatString=|
      | %<ID>
      | %<Vbase>V
      | %<VLF>pu
      | %<angleLF>deg.
      | %<Name>
  bus82 : powerlib/Measurements/Load Flow Bus  LConnTagsString=a  ID=bus82  Vbase=220000  Vref=1  Vangle=0  VLF=1  angleLF=0
      settings: AttributesFormatString=|
      | %<ID>
      | %<Vbase>V
      | %<VLF>pu
      | %<angleLF>deg.
      | %<Name>
  bus83 : powerlib/Measurements/Load Flow Bus  LConnTagsString=a  ID=bus83  Vbase=220000  Vref=1  Vangle=0  VLF=1  angleLF=0
      settings: AttributesFormatString=|
      | %<ID>
      | %<Vbase>V
      | %<VLF>pu
      | %<angleLF>deg.
      | %<Name>
  bus84 : powerlib/Measurements/Load Flow Bus  LConnTagsString=a  ID=bus84  Vbase=220000  Vref=1  Vangle=0  VLF=1  angleLF=0
      settings: AttributesFormatString=|
      | %<ID>
      | %<Vbase>V
      | %<VLF>pu
      | %<angleLF>deg.
      | %<Name>
  bus85 : powerlib/Measurements/Load Flow Bus  LConnTagsString=a  ID=bus85  Vbase=220000  Vref=1  Vangle=0  VLF=1  angleLF=0
      settings: AttributesFormatString=|
      | %<ID>
      | %<Vbase>V
      | %<VLF>pu
      | %<angleLF>deg.
      | %<Name>
  bus86 : powerlib/Measurements/Load Flow Bus  LConnTagsString=a  ID=bus86  Vbase=220000  Vref=1  Vangle=0  VLF=1  angleLF=0
      settings: AttributesFormatString=|
      | %<ID>
      | %<Vbase>V
      | %<VLF>pu
      | %<angleLF>deg.
      | %<Name>
  bus87 : powerlib/Measurements/Load Flow Bus  LConnTagsString=a  ID=bus87  Vbase=220000  Vref=1  Vangle=0  VLF=1  angleLF=0
      settings: AttributesFormatString=|
      | %<ID>
      | %<Vbase>V
      | %<VLF>pu
      | %<angleLF>deg.
      | %<Name>
  bus88 : powerlib/Measurements/Load Flow Bus  LConnTagsString=a  ID=bus88  Vbase=220000  Vref=1  Vangle=0  VLF=1  angleLF=0
      settings: AttributesFormatString=|
      | %<ID>
      | %<Vbase>V
      | %<VLF>pu
      | %<angleLF>deg.
      | %<Name>
  bus89 : powerlib/Measurements/Load Flow Bus  LConnTagsString=a  ID=bus89  Vbase=220000  Vref=1  Vangle=0  VLF=1  angleLF=0
      settings: AttributesFormatString=|
      | %<ID>
      | %<Vbase>V
      | %<VLF>pu
      | %<angleLF>deg.
      | %<Name>
  bus9 : powerlib/Measurements/Load Flow Bus  LConnTagsString=a  ID=bus9  Vbase=110000  Vref=1  Vangle=0  VLF=1  angleLF=0
      settings: AttributesFormatString=|
      | %<ID>
      | %<Vbase>V
      | %<VLF>pu
      | %<angleLF>deg.
      | %<Name>
  bus90 : powerlib/Measurements/Load Flow Bus  LConnTagsString=a  ID=bus90  Vbase=220000  Vref=1  Vangle=0  VLF=1  angleLF=0
      settings: AttributesFormatString=|
      | %<ID>
      | %<Vbase>V
      | %<VLF>pu
      | %<angleLF>deg.
      | %<Name>
  bus91 : powerlib/Measurements/Load Flow Bus  LConnTagsString=a  ID=bus91  Vbase=220000  Vref=1  Vangle=0  VLF=1  angleLF=0
      settings: AttributesFormatString=|
      | %<ID>
      | %<Vbase>V
      | %<VLF>pu
      | %<angleLF>deg.
      | %<Name>
  bus92 : powerlib/Measurements/Load Flow Bus  LConnTagsString=a  ID=bus92  Vbase=220000  Vref=1  Vangle=0  VLF=1  angleLF=0
      settings: AttributesFormatString=|
      | %<ID>
      | %<Vbase>V
      | %<VLF>pu
      | %<angleLF>deg.
      | %<Name>
  bus93 : powerlib/Measurements/Load Flow Bus  LConnTagsString=a  ID=bus93  Vbase=220000  Vref=1  Vangle=0  VLF=1  angleLF=0
      settings: AttributesFormatString=|
      | %<ID>
      | %<Vbase>V
      | %<VLF>pu
      | %<angleLF>deg.
      | %<Name>
  bus94 : powerlib/Measurements/Load Flow Bus  LConnTagsString=a  ID=bus94  Vbase=220000  Vref=1  Vangle=0  VLF=1  angleLF=0
      settings: AttributesFormatString=|
      | %<ID>
      | %<Vbase>V
      | %<VLF>pu
      | %<angleLF>deg.
      | %<Name>
  bus95 : powerlib/Measurements/Load Flow Bus  LConnTagsString=a  ID=bus95  Vbase=220000  Vref=1  Vangle=0  VLF=1  angleLF=0
      settings: AttributesFormatString=|
      | %<ID>
      | %<Vbase>V
      | %<VLF>pu
      | %<angleLF>deg.
      | %<Name>
  bus96 : powerlib/Measurements/Load Flow Bus  LConnTagsString=a  ID=bus96  Vbase=220000  Vref=1  Vangle=0  VLF=1  angleLF=0
      settings: AttributesFormatString=|
      | %<ID>
      | %<Vbase>V
      | %<VLF>pu
      | %<angleLF>deg.
      | %<Name>
  bus97 : powerlib/Measurements/Load Flow Bus  LConnTagsString=a  ID=bus97  Vbase=220000  Vref=1  Vangle=0  VLF=1  angleLF=0
      settings: AttributesFormatString=|
      | %<ID>
      | %<Vbase>V
      | %<VLF>pu
      | %<angleLF>deg.
      | %<Name>
  bus98 : powerlib/Measurements/Load Flow Bus  LConnTagsString=a  ID=bus98  Vbase=220000  Vref=1  Vangle=0  VLF=1  angleLF=0
      settings: AttributesFormatString=|
      | %<ID>
      | %<Vbase>V
      | %<VLF>pu
      | %<angleLF>deg.
      | %<Name>
  bus99 : powerlib/Measurements/Load Flow Bus  LConnTagsString=a  ID=bus99  Vbase=220000  Vref=1  Vangle=0  VLF=1  angleLF=0
      settings: AttributesFormatString=|
      | %<ID>
      | %<Vbase>V
      | %<VLF>pu
      | %<angleLF>deg.
      | %<Name>
  powergui : powerlib/powergui  Priority=1  SimulationMode=Continuous  SolverType=Tustin  SampleTime=50e-6  frequency=60  SPID=off  DisableSnubberDevices=off  DisableRonSwitches=off  DisableVfSwitches=off  SwTol=0  Interpol=off  DisplayEquations=off  Ts=0  methode=off  frequencyindice=60  Pbase=100e6  ErrMax=1e-4  Iterations=50  UnitsV=kV  UnitsW=MW  FunctionMessages=off  echomessages=off  HookPort=off  EnableUseOfTLC=off  x0status=blocks  RestoreLinks=warning  ResistiveCurrentMeasurement=off  Frange=[0:2:500]  Ylog=off  Xlog=on  ShowGrid=off  save=off  variable=ZData  structure=0  ZoomFFT=off  StartTime=0.0  cycles=1  DisplayStyle=1  fundamental=60  FreqAxis=off  MaxFrequency=1000  frequencyindicesteady=1  RmsSteady=1  display=off
  connections:
  _CN_161270797_110000_CN_95894638_110000/LConn1 -- T_161270797_220000;110000;33000_Albany_substation/RConn1 -- L_161270797/LConn1
  _CN_161270797_110000_CN_95894638_110000/LConn2 -- T_161270797_220000;110000;33000_Albany_substation/RConn2 -- L_161270797/LConn2
  _CN_161270797_110000_CN_95894638_110000/LConn3 -- T_161270797_220000;110000;33000_Albany_substation/RConn3 -- L_161270797/LConn3 -- bus1/LConn1
  _CN_161270797_110000_CN_95894638_110000/RConn1 -- T_95894638_220000;110000;33000_Wairau_Road_substation/RConn1 -- L_95894638/LConn1
  _CN_161270797_110000_CN_95894638_110000/RConn2 -- T_95894638_220000;110000;33000_Wairau_Road_substation/RConn2 -- L_95894638/LConn2
  _CN_161270797_110000_CN_95894638_110000/RConn3 -- T_95894638_220000;110000;33000_Wairau_Road_substation/RConn3 -- L_95894638/LConn3 -- bus2/LConn1
  T_400732687__/LConn1 -- _CN_400732687_110000_CN_173729963_110000/LConn1
  T_400732687__/LConn2 -- _CN_400732687_110000_CN_173729963_110000/LConn2
  _CN_400732687_110000_CN_173729963_110000/LConn3 -- T_400732687__/LConn3 -- bus3/LConn1
  T_173729963_110000;50000_Gisborne_substation/LConn1 -- _CN_400732687_110000_CN_173729963_110000/RConn1
  T_173729963_110000;50000_Gisborne_substation/LConn2 -- _CN_400732687_110000_CN_173729963_110000/RConn2
  _CN_400732687_110000_CN_173729963_110000/RConn3 -- T_173729963_110000;50000_Gisborne_substation/LConn3 -- bus4/LConn1
  T_167434770_110000;11000_Te_Awamutu_substation/LConn1 -- Karapiro_Te_Awamutu_110kV_CN_167434770_110000_CN_270536018_110000/LConn1
  T_167434770_110000;11000_Te_Awamutu_substation/LConn2 -- Karapiro_Te_Awamutu_110kV_CN_167434770_110000_CN_270536018_110000/LConn2
  Karapiro_Te_Awamutu_110kV_CN_167434770_110000_CN_270536018_110000/LConn3 -- T_167434770_110000;11000_Te_Awamutu_substation/LConn3 -- bus5/LConn1
  Karapiro_Te_Awamutu_110kV_CN_167434770_110000_CN_270536018_110000/RConn1 -- T_270536018_110000_Karapiro_substation/LConn1 -- Hinuera_Karapiro_110kV_CN_352911643_110000_CN_270536018_110000/LConn1 -- Hamilton_Karapiro_110kV_CN_340501677_110000_CN_270536018_110000/LConn1
  Karapiro_Te_Awamutu_110kV_CN_167434770_110000_CN_270536018_110000/RConn2 -- T_270536018_110000_Karapiro_substation/LConn2 -- Hinuera_Karapiro_110kV_CN_352911643_110000_CN_270536018_110000/LConn2 -- Hamilton_Karapiro_110kV_CN_340501677_110000_CN_270536018_110000/LConn2
  Karapiro_Te_Awamutu_110kV_CN_167434770_110000_CN_270536018_110000/RConn3 -- T_270536018_110000_Karapiro_substation/LConn3 -- Hinuera_Karapiro_110kV_CN_352911643_110000_CN_270536018_110000/LConn3 -- bus6/LConn1 -- Hamilton_Karapiro_110kV_CN_340501677_110000_CN_270536018_110000/LConn3
  Bunnythorpe_Ongarue_110kV_CN_167425043_110000_CN_410151576_110000/LConn1 -- T_167425043_110000;11000_Ohakune_substation/LConn1 -- Bunnythorpe_Ongarue_110kV_CN_167425043_110000_CN_367205270_110000/LConn1
  Bunnythorpe_Ongarue_110kV_CN_167425043_110000_CN_410151576_110000/LConn2 -- T_167425043_110000;11000_Ohakune_substation/LConn2 -- Bunnythorpe_Ongarue_110kV_CN_167425043_110000_CN_367205270_110000/LConn2
  Bunnythorpe_Ongarue_110kV_CN_167425043_110000_CN_410151576_110000/LConn3 -- T_167425043_110000;11000_Ohakune_substation/LConn3 -- Bunnythorpe_Ongarue_110kV_CN_167425043_110000_CN_367205270_110000/LConn3 -- bus7/LConn1
  Bunnythorpe_Ongarue_110kV_CN_167425043_110000_CN_410151576_110000/RConn1 -- T_410151576_110000;33000_Ongarue_substation/LConn1 -- _CN_410151576_110000_CN_272523195_110000/LConn1
  Bunnythorpe_Ongarue_110kV_CN_167425043_110000_CN_410151576_110000/RConn2 -- T_410151576_110000;33000_Ongarue_substation/LConn2 -- _CN_410151576_110000_CN_272523195_110000/LConn2
  Bunnythorpe_Ongarue_110kV_CN_167425043_110000_CN_410151576_110000/RConn3 -- T_410151576_110000;33000_Ongarue_substation/LConn3 -- _CN_410151576_110000_CN_272523195_110000/LConn3 -- bus8/LConn1
  Bunnythorpe_Ongarue_110kV_CN_167425043_110000_CN_367205270_110000/RConn1 -- T_367205270_110000;33000_Mataroa_substation/LConn1 -- Bunnythorpe_Ongarue_110kV_CN_167285336_110000_CN_367205270_110000/LConn1
  Bunnythorpe_Ongarue_110kV_CN_167425043_110000_CN_367205270_110000/RConn2 -- T_367205270_110000;33000_Mataroa_substation/LConn2 -- Bunnythorpe_Ongarue_110kV_CN_167285336_110000_CN_367205270_110000/LConn2
  Bunnythorpe_Ongarue_110kV_CN_167425043_110000_CN_367205270_110000/RConn3 -- T_367205270_110000;33000_Mataroa_substation/LConn3 -- Bunnythorpe_Ongarue_110kV_CN_167285336_110000_CN_367205270_110000/LConn3 -- bus9/LConn1
  T_168951331__Wheao_substation/LConn1 -- _CN_168951331_110000_CN_93844343_110000/LConn1
  T_168951331__Wheao_substation/LConn2 -- _CN_168951331_110000_CN_93844343_110000/LConn2
  _CN_168951331_110000_CN_93844343_110000/LConn3 -- T_168951331__Wheao_substation/LConn3 -- bus10/LConn1
  _CN_168951331_110000_CN_93844343_110000/RConn1 -- T_93844343_110000;33000;11000_Rotorua_substation/LConn1 -- Rotorua_Tarukenga_110kV_CN_93844343_110000_CN_270022030_110000/LConn1
  _CN_168951331_110000_CN_93844343_110000/RConn2 -- T_93844343_110000;33000;11000_Rotorua_substation/LConn2 -- Rotorua_Tarukenga_110kV_CN_93844343_110000_CN_270022030_110000/LConn2
  _CN_168951331_110000_CN_93844343_110000/RConn3 -- T_93844343_110000;33000;11000_Rotorua_substation/LConn3 -- Rotorua_Tarukenga_110kV_CN_93844343_110000_CN_270022030_110000/LConn3 -- bus11/LConn1
  _CN_232293420_110000_CN_413551915_110000/LConn1 -- T_232293420_110000_Tuai_substation/LConn1 -- _CN_232293420_110000_CN_93419961_110000/LConn1
  _CN_232293420_110000_CN_413551915_110000/LConn2 -- T_232293420_110000_Tuai_substation/LConn2 -- _CN_232293420_110000_CN_93419961_110000/LConn2
  _CN_232293420_110000_CN_413551915_110000/LConn3 -- T_232293420_110000_Tuai_substation/LConn3 -- _CN_232293420_110000_CN_93419961_110000/LConn3 -- bus12/LConn1
  T_413551915_110000;50000;33000;11000_Wairoa_substation/LConn1 -- _CN_232293420_110000_CN_413551915_110000/RConn1
  T_413551915_110000;50000;33000;11000_Wairoa_substation/LConn2 -- _CN_232293420_110000_CN_413551915_110000/RConn2
  _CN_232293420_110000_CN_413551915_110000/RConn3 -- T_413551915_110000;50000;33000;11000_Wairoa_substation/LConn3 -- bus13/LConn1
  _CN_232293420_110000_CN_93419961_110000/RConn1 -- T_93419961_110000;33000_Fernhill_substation/LConn1 -- _CN_168096434_110000_CN_93419961_110000/LConn1
  _CN_232293420_110000_CN_93419961_110000/RConn2 -- T_93419961_110000;33000_Fernhill_substation/LConn2 -- _CN_168096434_110000_CN_93419961_110000/LConn2
  _CN_232293420_110000_CN_93419961_110000/RConn3 -- T_93419961_110000;33000_Fernhill_substation/LConn3 -- _CN_168096434_110000_CN_93419961_110000/LConn3 -- bus14/LConn1
  T_187865148_110000;33000_Hangatiki_substation/LConn1 -- _CN_187865148_110000_CN_272523195_110000/LConn1
  T_187865148_110000;33000_Hangatiki_substation/LConn2 -- _CN_187865148_110000_CN_272523195_110000/LConn2
  _CN_187865148_110000_CN_272523195_110000/LConn3 -- T_187865148_110000;33000_Hangatiki_substation/LConn3 -- bus15/LConn1
  _CN_187865148_110000_CN_272523195_110000/RConn1 -- T_272523195_110000_Arapuni_substation/LConn1 -- _CN_140103942_110000_CN_272523195_110000/LConn1 -- _CN_410151576_110000_CN_272523195_110000/RConn1
  _CN_187865148_110000_CN_272523195_110000/RConn2 -- T_272523195_110000_Arapuni_substation/LConn2 -- _CN_140103942_110000_CN_272523195_110000/LConn2 -- _CN_410151576_110000_CN_272523195_110000/RConn2
  _CN_187865148_110000_CN_272523195_110000/RConn3 -- T_272523195_110000_Arapuni_substation/LConn3 -- _CN_140103942_110000_CN_272523195_110000/LConn3 -- bus16/LConn1 -- _CN_410151576_110000_CN_272523195_110000/RConn3
  T_168231493_110000_Inangahua_substation/LConn1 -- _CN_168231493_110000_CN_231527208_110000/LConn1
  T_168231493_110000_Inangahua_substation/LConn2 -- _CN_168231493_110000_CN_231527208_110000/LConn2
  _CN_168231493_110000_CN_231527208_110000/LConn3 -- T_168231493_110000_Inangahua_substation/LConn3 -- bus17/LConn1
  T_231527208__/LConn1 -- _CN_168231493_110000_CN_231527208_110000/RConn1
  T_231527208__/LConn2 -- _CN_168231493_110000_CN_231527208_110000/RConn2
  _CN_168231493_110000_CN_231527208_110000/RConn3 -- T_231527208__/LConn3 -- bus18/LConn1
  T_90092619_110000;33000_Edendale_substation/LConn1 -- Gore_Invercargill_110kV_CN_90092619_110000_CN_224937549_110000/LConn1
  T_90092619_110000;33000_Edendale_substation/LConn2 -- Gore_Invercargill_110kV_CN_90092619_110000_CN_224937549_110000/LConn2
  Gore_Invercargill_110kV_CN_90092619_110000_CN_224937549_110000/LConn3 -- T_90092619_110000;33000_Edendale_substation/LConn3 -- bus19/LConn1
  T_224937549_110000_Brydone_substation/LConn1 -- Gore_Invercargill_110kV_CN_90092619_110000_CN_224937549_110000/RConn1
  T_224937549_110000_Brydone_substation/LConn2 -- Gore_Invercargill_110kV_CN_90092619_110000_CN_224937549_110000/RConn2
  Gore_Invercargill_110kV_CN_90092619_110000_CN_224937549_110000/RConn3 -- T_224937549_110000_Brydone_substation/LConn3 -- bus20/LConn1
  Bunnythorpe_Ongarue_110kV_CN_167285336_110000_CN_367205270_110000/RConn1 -- T_167285336_220000;110000;50000;33000_Bunnythorpe_substation/RConn1 -- L_167285336/LConn1
  Bunnythorpe_Ongarue_110kV_CN_167285336_110000_CN_367205270_110000/RConn2 -- T_167285336_220000;110000;50000;33000_Bunnythorpe_substation/RConn2 -- L_167285336/LConn2
  Bunnythorpe_Ongarue_110kV_CN_167285336_110000_CN_367205270_110000/RConn3 -- T_167285336_220000;110000;50000;33000_Bunnythorpe_substation/RConn3 -- L_167285336/LConn3 -- bus21/LConn1
  _CN_87338082_110000_CN_270022030_110000/LConn1 -- T_87338082_110000_Lichfield_substation/LConn1 -- _CN_87338082_110000_CN_140103942_110000/LConn1
  _CN_87338082_110000_CN_270022030_110000/LConn2 -- T_87338082_110000_Lichfield_substation/LConn2 -- _CN_87338082_110000_CN_140103942_110000/LConn2
  _CN_87338082_110000_CN_270022030_110000/LConn3 -- T_87338082_110000_Lichfield_substation/LConn3 -- _CN_87338082_110000_CN_140103942_110000/LConn3 -- bus22/LConn1
  _CN_87338082_110000_CN_270022030_110000/RConn1 -- T_270022030_220000;110000;11000_Tarukenga_substation/RConn1 -- Rotorua_Tarukenga_110kV_CN_93844343_110000_CN_270022030_110000/RConn1 -- _CN_93707134_110000_CN_270022030_110000/LConn1 -- L_270022030/LConn1
  _CN_87338082_110000_CN_270022030_110000/RConn2 -- T_270022030_220000;110000;11000_Tarukenga_substation/RConn2 -- Rotorua_Tarukenga_110kV_CN_93844343_110000_CN_270022030_110000/RConn2 -- _CN_93707134_110000_CN_270022030_110000/LConn2 -- L_270022030/LConn2
  _CN_87338082_110000_CN_270022030_110000/RConn3 -- T_270022030_220000;110000;11000_Tarukenga_substation/RConn3 -- Rotorua_Tarukenga_110kV_CN_93844343_110000_CN_270022030_110000/RConn3 -- _CN_93707134_110000_CN_270022030_110000/LConn3 -- L_270022030/LConn3 -- bus23/LConn1
  _CN_87338082_110000_CN_140103942_110000/RConn1 -- T_140103942__/LConn1 -- _CN_140103942_110000_CN_272523195_110000/RConn1
  _CN_87338082_110000_CN_140103942_110000/RConn2 -- T_140103942__/LConn2 -- _CN_140103942_110000_CN_272523195_110000/RConn2
  _CN_87338082_110000_CN_140103942_110000/RConn3 -- T_140103942__/LConn3 -- _CN_140103942_110000_CN_272523195_110000/RConn3 -- bus24/LConn1
  Waihou_Waikino_110kV_CN_174382184_110000_CN_87894783_110000/LConn1 -- T_174382184_110000;33000_Waikino_substation/LConn1 -- Kopu_Waikino_110kV_CN_174382184_110000_CN_146612611_110000/LConn1
  Waihou_Waikino_110kV_CN_174382184_110000_CN_87894783_110000/LConn2 -- T_174382184_110000;33000_Waikino_substation/LConn2 -- Kopu_Waikino_110kV_CN_174382184_110000_CN_146612611_110000/LConn2
  Waihou_Waikino_110kV_CN_174382184_110000_CN_87894783_110000/LConn3 -- T_174382184_110000;33000_Waikino_substation/LConn3 -- Kopu_Waikino_110kV_CN_174382184_110000_CN_146612611_110000/LConn3 -- bus25/LConn1
  Waihou_Waikino_110kV_CN_174382184_110000_CN_87894783_110000/RConn1 -- T_87894783_110000;33000_Waihou_substation/LConn1 -- Hamilton_Waihou_110kV_CN_87894783_110000_CN_94053861_110000/LConn1
  Waihou_Waikino_110kV_CN_174382184_110000_CN_87894783_110000/RConn2 -- T_87894783_110000;33000_Waihou_substation/LConn2 -- Hamilton_Waihou_110kV_CN_87894783_110000_CN_94053861_110000/LConn2
  Waihou_Waikino_110kV_CN_174382184_110000_CN_87894783_110000/RConn3 -- T_87894783_110000;33000_Waihou_substation/LConn3 -- Hamilton_Waihou_110kV_CN_87894783_110000_CN_94053861_110000/LConn3 -- bus26/LConn1
  T_146612611_110000;66000_Kopu_substation/LConn1 -- Kopu_Waikino_110kV_CN_174382184_110000_CN_146612611_110000/RConn1
  T_146612611_110000;66000_Kopu_substation/LConn2 -- Kopu_Waikino_110kV_CN_174382184_110000_CN_146612611_110000/RConn2
  Kopu_Waikino_110kV_CN_174382184_110000_CN_146612611_110000/RConn3 -- T_146612611_110000;66000_Kopu_substation/LConn3 -- bus27/LConn1
  T_218862188_110000;33000_Balclutha_substation/LConn1 -- Balclutha_deviation_110kV_CN_218862188_110000_CN_413796046_110000/LConn1
  T_218862188_110000;33000_Balclutha_substation/LConn2 -- Balclutha_deviation_110kV_CN_218862188_110000_CN_413796046_110000/LConn2
  Balclutha_deviation_110kV_CN_218862188_110000_CN_413796046_110000/LConn3 -- T_218862188_110000;33000_Balclutha_substation/LConn3 -- bus28/LConn1
  T_413796046_110000_Berwick_substation/LConn1 -- Balclutha_deviation_110kV_CN_218862188_110000_CN_413796046_110000/RConn1
  T_413796046_110000_Berwick_substation/LConn2 -- Balclutha_deviation_110kV_CN_218862188_110000_CN_413796046_110000/RConn2
  Balclutha_deviation_110kV_CN_218862188_110000_CN_413796046_110000/RConn3 -- T_413796046_110000_Berwick_substation/LConn3 -- bus29/LConn1
  Henderson_Hepburn_Road_CN_26671244_110000_CN_51867062_110000/LConn1 -- T_26671244_220000;110000;33000_Henderson_substation/RConn1 -- Henderson_Maungatapere_110kV_CN_26671244_110000_CN_168228811_110000/LConn1 -- L_26671244/LConn1
  Henderson_Hepburn_Road_CN_26671244_110000_CN_51867062_110000/LConn2 -- T_26671244_220000;110000;33000_Henderson_substation/RConn2 -- Henderson_Maungatapere_110kV_CN_26671244_110000_CN_168228811_110000/LConn2 -- L_26671244/LConn2
  Henderson_Hepburn_Road_CN_26671244_110000_CN_51867062_110000/LConn3 -- T_26671244_220000;110000;33000_Henderson_substation/RConn3 -- Henderson_Maungatapere_110kV_CN_26671244_110000_CN_168228811_110000/LConn3 -- L_26671244/LConn3 -- bus30/LConn1
  Henderson_Hepburn_Road_CN_26671244_110000_CN_51867062_110000/RConn1 -- T_51867062_110000;33000_Hepburn_Road_substation/LConn1 -- _CN_27030962_110000_CN_51867062_110000/LConn1
  Henderson_Hepburn_Road_CN_26671244_110000_CN_51867062_110000/RConn2 -- T_51867062_110000;33000_Hepburn_Road_substation/LConn2 -- _CN_27030962_110000_CN_51867062_110000/LConn2
  Henderson_Hepburn_Road_CN_26671244_110000_CN_51867062_110000/RConn3 -- T_51867062_110000;33000_Hepburn_Road_substation/LConn3 -- _CN_27030962_110000_CN_51867062_110000/LConn3 -- bus31/LConn1
  Henderson_Maungatapere_110kV_CN_26671244_110000_CN_168228811_110000/RConn1 -- T_168228811__Wellsford_substation/LConn1 -- _CN_168228811_110000_CN_193039355_110000/LConn1
  Henderson_Maungatapere_110kV_CN_26671244_110000_CN_168228811_110000/RConn2 -- T_168228811__Wellsford_substation/LConn2 -- _CN_168228811_110000_CN_193039355_110000/LConn2
  Henderson_Maungatapere_110kV_CN_26671244_110000_CN_168228811_110000/RConn3 -- T_168228811__Wellsford_substation/LConn3 -- _CN_168228811_110000_CN_193039355_110000/LConn3 -- bus32/LConn1
  T_93836457_110000;33000_Huirangi_substation/LConn1 -- Carrington_Street_Huirangi_110kV_CN_93836457_110000_CN_93836458_110000/LConn1
  T_93836457_110000;33000_Huirangi_substation/LConn2 -- Carrington_Street_Huirangi_110kV_CN_93836457_110000_CN_93836458_110000/LConn2
  Carrington_Street_Huirangi_110kV_CN_93836457_110000_CN_93836458_110000/LConn3 -- T_93836457_110000;33000_Huirangi_substation/LConn3 -- bus33/LConn1
  Carrington_Street_Huirangi_110kV_CN_93836457_110000_CN_93836458_110000/RConn1 -- T_93836458_110000;33000_Carrington_Street_substation/LConn1 -- Carrington_Street_New_Plymouth_110kV_CN_93836463_110000_CN_93836458_110000/LConn1
  Carrington_Street_Huirangi_110kV_CN_93836457_110000_CN_93836458_110000/RConn2 -- T_93836458_110000;33000_Carrington_Street_substation/LConn2 -- Carrington_Street_New_Plymouth_110kV_CN_93836463_110000_CN_93836458_110000/LConn2
  Carrington_Street_Huirangi_110kV_CN_93836457_110000_CN_93836458_110000/RConn3 -- T_93836458_110000;33000_Carrington_Street_substation/LConn3 -- Carrington_Street_New_Plymouth_110kV_CN_93836463_110000_CN_93836458_110000/LConn3 -- bus34/LConn1
  Hamilton_Karapiro_110kV_CN_340501677_110000_CN_94053861_110000/LConn1 -- T_340501677_110000;11000_Cambridge_substation/LConn1 -- Hamilton_Karapiro_110kV_CN_340501677_110000_CN_270536018_110000/RConn1
  Hamilton_Karapiro_110kV_CN_340501677_110000_CN_94053861_110000/LConn2 -- T_340501677_110000;11000_Cambridge_substation/LConn2 -- Hamilton_Karapiro_110kV_CN_340501677_110000_CN_270536018_110000/RConn2
  Hamilton_Karapiro_110kV_CN_340501677_110000_CN_94053861_110000/LConn3 -- T_340501677_110000;11000_Cambridge_substation/LConn3 -- Hamilton_Karapiro_110kV_CN_340501677_110000_CN_270536018_110000/RConn3 -- bus35/LConn1
  Hamilton_Karapiro_110kV_CN_340501677_110000_CN_94053861_110000/RConn1 -- T_94053861_220000;110000;55000;33000;11000_Hamilton_sub_station/LConn1 -- Hamilton_Waihou_110kV_CN_87894783_110000_CN_94053861_110000/RConn1
  Hamilton_Karapiro_110kV_CN_340501677_110000_CN_94053861_110000/RConn2 -- T_94053861_220000;110000;55000;33000;11000_Hamilton_sub_station/LConn2 -- Hamilton_Waihou_110kV_CN_87894783_110000_CN_94053861_110000/RConn2
  Hamilton_Karapiro_110kV_CN_340501677_110000_CN_94053861_110000/RConn3 -- T_94053861_220000;110000;55000;33000;11000_Hamilton_sub_station/LConn3 -- Hamilton_Waihou_110kV_CN_87894783_110000_CN_94053861_110000/RConn3 -- bus36/LConn1
  T_93836463_220000;110000;33000_New_Plymouth_substation/LConn1 -- Carrington_Street_New_Plymouth_110kV_CN_93836463_110000_CN_93836458_110000/RConn1
  T_93836463_220000;110000;33000_New_Plymouth_substation/LConn2 -- Carrington_Street_New_Plymouth_110kV_CN_93836463_110000_CN_93836458_110000/RConn2
  Carrington_Street_New_Plymouth_110kV_CN_93836463_110000_CN_93836458_110000/RConn3 -- T_93836463_220000;110000;33000_New_Plymouth_substation/LConn3 -- bus37/LConn1
  _CN_168096434_110000_CN_367194918_110000/LConn1 -- T_168096434_110000;33000;11000_Waipawa_substation/LConn1 -- _CN_168096434_110000_CN_93419961_110000/RConn1
  _CN_168096434_110000_CN_367194918_110000/LConn2 -- T_168096434_110000;33000;11000_Waipawa_substation/LConn2 -- _CN_168096434_110000_CN_93419961_110000/RConn2
  _CN_168096434_110000_CN_367194918_110000/LConn3 -- T_168096434_110000;33000;11000_Waipawa_substation/LConn3 -- _CN_168096434_110000_CN_93419961_110000/RConn3 -- bus38/LConn1
  _CN_168096434_110000_CN_367194918_110000/RConn1 -- T_367194918_110000;11000_Dannevirke_substation/LConn1 -- Fernhill_Woodville_B_CN_367194918_110000_CN_269748077_110000/LConn1
  _CN_168096434_110000_CN_367194918_110000/RConn2 -- T_367194918_110000;11000_Dannevirke_substation/LConn2 -- Fernhill_Woodville_B_CN_367194918_110000_CN_269748077_110000/LConn2
  _CN_168096434_110000_CN_367194918_110000/RConn3 -- T_367194918_110000;11000_Dannevirke_substation/LConn3 -- Fernhill_Woodville_B_CN_367194918_110000_CN_269748077_110000/LConn3 -- bus39/LConn1
  T_180636348_110000;33000_Kensington_substation/LConn1 -- Kensington_Maungatapere_110kV_CN_180636348_110000_CN_101442986_110000/LConn1
  T_180636348_110000;33000_Kensington_substation/LConn2 -- Kensington_Maungatapere_110kV_CN_180636348_110000_CN_101442986_110000/LConn2
  Kensington_Maungatapere_110kV_CN_180636348_110000_CN_101442986_110000/LConn3 -- T_180636348_110000;33000_Kensington_substation/LConn3 -- bus40/LConn1
  Kensington_Maungatapere_110kV_CN_180636348_110000_CN_101442986_110000/RConn1 -- T_101442986_110000;50000;33000_Maungatapere_substation/LConn1 -- _CN_167952087_110000_CN_101442986_110000/LConn1
  Kensington_Maungatapere_110kV_CN_180636348_110000_CN_101442986_110000/RConn2 -- T_101442986_110000;50000;33000_Maungatapere_substation/LConn2 -- _CN_167952087_110000_CN_101442986_110000/LConn2
  Kensington_Maungatapere_110kV_CN_180636348_110000_CN_101442986_110000/RConn3 -- T_101442986_110000;50000;33000_Maungatapere_substation/LConn3 -- _CN_167952087_110000_CN_101442986_110000/LConn3 -- bus41/LConn1
  _CN_97334973_110000_CN_160708893_110000/LConn1 -- T_97334973_110000;33000_Mount_Maunganui_substation/LConn1 -- _CN_97334973_110000_CN_119877500_110000/LConn1
  _CN_97334973_110000_CN_160708893_110000/LConn2 -- T_97334973_110000;33000_Mount_Maunganui_substation/LConn2 -- _CN_97334973_110000_CN_119877500_110000/LConn2
  _CN_97334973_110000_CN_160708893_110000/LConn3 -- T_97334973_110000;33000_Mount_Maunganui_substation/LConn3 -- _CN_97334973_110000_CN_119877500_110000/LConn3 -- bus42/LConn1
  T_160708893_110000;33000_Tauranga_substation/LConn1 -- _CN_97334973_110000_CN_160708893_110000/RConn1
  T_160708893_110000;33000_Tauranga_substation/LConn2 -- _CN_97334973_110000_CN_160708893_110000/RConn2
  _CN_97334973_110000_CN_160708893_110000/RConn3 -- T_160708893_110000;33000_Tauranga_substation/LConn3 -- bus43/LConn1
  _CN_97334973_110000_CN_119877500_110000/RConn1 -- T_119877500_220000;110000;33000_Kaitimako_sub_station/LConn1 -- _CN_161010976_110000_CN_119877500_110000/LConn1
  _CN_97334973_110000_CN_119877500_110000/RConn2 -- T_119877500_220000;110000;33000_Kaitimako_sub_station/LConn2 -- _CN_161010976_110000_CN_119877500_110000/LConn2
  _CN_97334973_110000_CN_119877500_110000/RConn3 -- T_119877500_220000;110000;33000_Kaitimako_sub_station/LConn3 -- _CN_161010976_110000_CN_119877500_110000/LConn3 -- bus44/LConn1
  Mangere_Otahuhu_110kV_CN_75609279_110000_CN_410455856_110000/LConn1 -- T_75609279_220000;110000_Otahuhu_substation/RConn1 -- L_75609279/LConn1
  Mangere_Otahuhu_110kV_CN_75609279_110000_CN_410455856_110000/LConn2 -- T_75609279_220000;110000_Otahuhu_substation/RConn2 -- L_75609279/LConn2
  Mangere_Otahuhu_110kV_CN_75609279_110000_CN_410455856_110000/LConn3 -- T_75609279_220000;110000_Otahuhu_substation/RConn3 -- L_75609279/LConn3 -- bus45/LConn1
  T_410455856_110000;33000_Mangere_substation/LConn1 -- Mangere_Otahuhu_110kV_CN_75609279_110000_CN_410455856_110000/RConn1
  T_410455856_110000;33000_Mangere_substation/LConn2 -- Mangere_Otahuhu_110kV_CN_75609279_110000_CN_410455856_110000/RConn2
  Mangere_Otahuhu_110kV_CN_75609279_110000_CN_410455856_110000/RConn3 -- T_410455856_110000;33000_Mangere_substation/LConn3 -- bus46/LConn1
  T_269746976_110000;33000_Masterton_substation/LConn1 -- _CN_269746976_110000_CN_167285978_110000/LConn1
  T_269746976_110000;33000_Masterton_substation/LConn2 -- _CN_269746976_110000_CN_167285978_110000/LConn2
  _CN_269746976_110000_CN_167285978_110000/LConn3 -- T_269746976_110000;33000_Masterton_substation/LConn3 -- bus47/LConn1
  _CN_269746976_110000_CN_167285978_110000/RConn1 -- T_167285978_110000;33000_Mangamaire_substation/LConn1 -- Mangamaire_Woodville_110kV_CN_167285978_110000_CN_269748077_110000/LConn1
  _CN_269746976_110000_CN_167285978_110000/RConn2 -- T_167285978_110000;33000_Mangamaire_substation/LConn2 -- Mangamaire_Woodville_110kV_CN_167285978_110000_CN_269748077_110000/LConn2
  _CN_269746976_110000_CN_167285978_110000/RConn3 -- T_167285978_110000;33000_Mangamaire_substation/LConn3 -- Mangamaire_Woodville_110kV_CN_167285978_110000_CN_269748077_110000/LConn3 -- bus48/LConn1
  T_25176792_110000;33000;11000_Central_Park_substation/LConn1 -- _CN_25176792_110000_CN_95343089_110000/LConn1
  T_25176792_110000;33000;11000_Central_Park_substation/LConn2 -- _CN_25176792_110000_CN_95343089_110000/LConn2
  _CN_25176792_110000_CN_95343089_110000/LConn3 -- T_25176792_110000;33000;11000_Central_Park_substation/LConn3 -- bus49/LConn1
  _CN_25176792_110000_CN_95343089_110000/RConn1 -- T_95343089_220000;110000;33000_Wilton_substation/LConn1 -- Takapu_Road_Wilton_110kV_CN_95343088_110000_CN_95343089_110000/LConn1
  _CN_25176792_110000_CN_95343089_110000/RConn2 -- T_95343089_220000;110000;33000_Wilton_substation/LConn2 -- Takapu_Road_Wilton_110kV_CN_95343088_110000_CN_95343089_110000/LConn2
  _CN_25176792_110000_CN_95343089_110000/RConn3 -- T_95343089_220000;110000;33000_Wilton_substation/LConn3 -- Takapu_Road_Wilton_110kV_CN_95343088_110000_CN_95343089_110000/LConn3 -- bus50/LConn1
  Mangamaire_Woodville_110kV_CN_167285978_110000_CN_269748077_110000/RConn1 -- T_269748077_110000;11000_Woodville_substation/LConn1 -- Te_Apiti_Woodville_110kV_CN_269748077_110000_CN_269748078_110000/LConn1 -- Fernhill_Woodville_B_CN_367194918_110000_CN_269748077_110000/RConn1
  Mangamaire_Woodville_110kV_CN_167285978_110000_CN_269748077_110000/RConn2 -- T_269748077_110000;11000_Woodville_substation/LConn2 -- Te_Apiti_Woodville_110kV_CN_269748077_110000_CN_269748078_110000/LConn2 -- Fernhill_Woodville_B_CN_367194918_110000_CN_269748077_110000/RConn2
  Mangamaire_Woodville_110kV_CN_167285978_110000_CN_269748077_110000/RConn3 -- T_269748077_110000;11000_Woodville_substation/LConn3 -- Te_Apiti_Woodville_110kV_CN_269748077_110000_CN_269748078_110000/LConn3 -- bus51/LConn1 -- Fernhill_Woodville_B_CN_367194918_110000_CN_269748077_110000/RConn3
  Haywards_Melling_110kV_CN_93713115_110000_CN_29545850_110000/LConn1 -- T_93713115_350000;220000_Haywards_static_inverter_plant/RConn1 -- L_93713115/LConn1
  Haywards_Melling_110kV_CN_93713115_110000_CN_29545850_110000/LConn2 -- T_93713115_350000;220000_Haywards_static_inverter_plant/RConn2 -- L_93713115/LConn2
  Haywards_Melling_110kV_CN_93713115_110000_CN_29545850_110000/LConn3 -- T_93713115_350000;220000_Haywards_static_inverter_plant/RConn3 -- L_93713115/LConn3 -- bus52/LConn1
  T_29545850_110000;33000;11000_Melling_substation/LConn1 -- Haywards_Melling_110kV_CN_93713115_110000_CN_29545850_110000/RConn1
  T_29545850_110000;33000;11000_Melling_substation/LConn2 -- Haywards_Melling_110kV_CN_93713115_110000_CN_29545850_110000/RConn2
  Haywards_Melling_110kV_CN_93713115_110000_CN_29545850_110000/RConn3 -- T_29545850_110000;33000;11000_Melling_substation/LConn3 -- bus53/LConn1
  T_260242665_110000;22000_Kingsland_zone_substation/LConn1 -- _CN_260242665_110000_CN_27030962_110000/LConn1
  T_260242665_110000;22000_Kingsland_zone_substation/LConn2 -- _CN_260242665_110000_CN_27030962_110000/LConn2
  _CN_260242665_110000_CN_27030962_110000/LConn3 -- T_260242665_110000;22000_Kingsland_zone_substation/LConn3 -- bus54/LConn1
  _CN_260242665_110000_CN_27030962_110000/RConn1 -- T_27030962_110000;22000_Mount_Roskill_substation/LConn1 -- Mangere_Mount_Roskill_110kV;_Mount_Roskill_Otahuhu_110kV;_Mount_Roskill_Otahuhu_110kV_CN_27030962_110000_CN_363290611_110000/LConn1 -- _CN_154965833_110000_CN_27030962_110000/LConn1 -- _CN_27030962_110000_CN_51867062_110000/RConn1
  _CN_260242665_110000_CN_27030962_110000/RConn2 -- T_27030962_110000;22000_Mount_Roskill_substation/LConn2 -- Mangere_Mount_Roskill_110kV;_Mount_Roskill_Otahuhu_110kV;_Mount_Roskill_Otahuhu_110kV_CN_27030962_110000_CN_363290611_110000/LConn2 -- _CN_154965833_110000_CN_27030962_110000/LConn2 -- _CN_27030962_110000_CN_51867062_110000/RConn2
  _CN_260242665_110000_CN_27030962_110000/RConn3 -- T_27030962_110000;22000_Mount_Roskill_substation/LConn3 -- Mangere_Mount_Roskill_110kV;_Mount_Roskill_Otahuhu_110kV;_Mount_Roskill_Otahuhu_110kV_CN_27030962_110000_CN_363290611_110000/LConn3 -- bus55/LConn1 -- _CN_154965833_110000_CN_27030962_110000/LConn3 -- _CN_27030962_110000_CN_51867062_110000/RConn3
  T_167952087_110000_Kaikohe_substation/LConn1 -- _CN_167952087_110000_CN_101442986_110000/RConn1
  T_167952087_110000_Kaikohe_substation/LConn2 -- _CN_167952087_110000_CN_101442986_110000/RConn2
  _CN_167952087_110000_CN_101442986_110000/RConn3 -- T_167952087_110000_Kaikohe_substation/LConn3 -- bus56/LConn1
  T_352911643_110000;33000_Hineura_substation/LConn1 -- Hinuera_Karapiro_110kV_CN_352911643_110000_CN_270536018_110000/RConn1
  T_352911643_110000;33000_Hineura_substation/LConn2 -- Hinuera_Karapiro_110kV_CN_352911643_110000_CN_270536018_110000/RConn2
  Hinuera_Karapiro_110kV_CN_352911643_110000_CN_270536018_110000/RConn3 -- T_352911643_110000;33000_Hineura_substation/LConn3 -- bus57/LConn1
  T_161010976_110000;33000_Te_Matai_substation/LConn1 -- _CN_161010976_110000_CN_119877500_110000/RConn1
  T_161010976_110000;33000_Te_Matai_substation/LConn2 -- _CN_161010976_110000_CN_119877500_110000/RConn2
  _CN_161010976_110000_CN_119877500_110000/RConn3 -- T_161010976_110000;33000_Te_Matai_substation/LConn3 -- bus58/LConn1
  _CN_154965833_110000_CN_87495237_110000/LConn1 -- T_154965833_110000;22000_Liverpool_zone_substation/LConn1 -- _CN_154965833_110000_CN_158810608_110000/LConn1 -- _CN_154965833_110000_CN_156097401_110000/LConn1 -- _CN_154965833_110000_CN_27030962_110000/RConn1
  _CN_154965833_110000_CN_87495237_110000/LConn2 -- T_154965833_110000;22000_Liverpool_zone_substation/LConn2 -- _CN_154965833_110000_CN_158810608_110000/LConn2 -- _CN_154965833_110000_CN_156097401_110000/LConn2 -- _CN_154965833_110000_CN_27030962_110000/RConn2
  _CN_154965833_110000_CN_87495237_110000/LConn3 -- T_154965833_110000;22000_Liverpool_zone_substation/LConn3 -- _CN_154965833_110000_CN_158810608_110000/LConn3 -- bus59/LConn1 -- _CN_154965833_110000_CN_156097401_110000/LConn3 -- _CN_154965833_110000_CN_27030962_110000/RConn3
  _CN_154965833_110000_CN_87495237_110000/RConn1 -- T_87495237_110000_Penrose_substation_(110kV)/LConn1 -- Otahuhu_Penrose_110kV_CN_87495237_110000_CN_363290611_110000/LConn1 -- _CN_87495237_110000_CN_359449581_110000/LConn1
  _CN_154965833_110000_CN_87495237_110000/RConn2 -- T_87495237_110000_Penrose_substation_(110kV)/LConn2 -- Otahuhu_Penrose_110kV_CN_87495237_110000_CN_363290611_110000/LConn2 -- _CN_87495237_110000_CN_359449581_110000/LConn2
  _CN_154965833_110000_CN_87495237_110000/RConn3 -- T_87495237_110000_Penrose_substation_(110kV)/LConn3 -- Otahuhu_Penrose_110kV_CN_87495237_110000_CN_363290611_110000/LConn3 -- _CN_87495237_110000_CN_359449581_110000/LConn3 -- bus60/LConn1
  _CN_154965833_110000_CN_156097401_110000/RConn1 -- T_156097401_220000;110000;22000;11000_Hobson_Street_substation/RConn1 -- L_156097401/LConn1
  _CN_154965833_110000_CN_156097401_110000/RConn2 -- T_156097401_220000;110000;22000;11000_Hobson_Street_substation/RConn2 -- L_156097401/LConn2
  _CN_154965833_110000_CN_156097401_110000/RConn3 -- T_156097401_220000;110000;22000;11000_Hobson_Street_substation/RConn3 -- L_156097401/LConn3 -- bus61/LConn1
  T_158810608_110000;22000;11000_Quay_zone_substation/LConn1 -- _CN_154965833_110000_CN_158810608_110000/RConn1
  T_158810608_110000;22000;11000_Quay_zone_substation/LConn2 -- _CN_154965833_110000_CN_158810608_110000/RConn2
  _CN_154965833_110000_CN_158810608_110000/RConn3 -- T_158810608_110000;22000;11000_Quay_zone_substation/LConn3 -- bus62/LConn1
  T_272196494_110000;33000_Blenheim_substation/LConn1 -- Blenheim_Stoke_CN_272196494_110000_CN_167705537_110000/LConn1
  T_272196494_110000;33000_Blenheim_substation/LConn2 -- Blenheim_Stoke_CN_272196494_110000_CN_167705537_110000/LConn2
  Blenheim_Stoke_CN_272196494_110000_CN_167705537_110000/LConn3 -- T_272196494_110000;33000_Blenheim_substation/LConn3 -- bus63/LConn1
  T_167705537_220000;110000;66000;33000_Stoke_substation/LConn1 -- Blenheim_Stoke_CN_272196494_110000_CN_167705537_110000/RConn1
  T_167705537_220000;110000;66000;33000_Stoke_substation/LConn2 -- Blenheim_Stoke_CN_272196494_110000_CN_167705537_110000/RConn2
  Blenheim_Stoke_CN_272196494_110000_CN_167705537_110000/RConn3 -- T_167705537_220000;110000;66000;33000_Stoke_substation/LConn3 -- bus64/LConn1
  T_182456667_110000_/LConn1 -- _CN_182456667_110000_CN_182466629_110000/LConn1
  T_182456667_110000_/LConn2 -- _CN_182456667_110000_CN_182466629_110000/LConn2
  _CN_182456667_110000_CN_182466629_110000/LConn3 -- T_182456667_110000_/LConn3 -- bus65/LConn1
  T_182466629__/LConn1 -- _CN_182456667_110000_CN_182466629_110000/RConn1
  T_182466629__/LConn2 -- _CN_182456667_110000_CN_182466629_110000/RConn2
  _CN_182456667_110000_CN_182466629_110000/RConn3 -- T_182466629__/LConn3 -- bus66/LConn1
  T_269748078_110000_Te_Apiti_substation/LConn1 -- Te_Apiti_Woodville_110kV_CN_269748077_110000_CN_269748078_110000/RConn1
  T_269748078_110000_Te_Apiti_substation/LConn2 -- Te_Apiti_Woodville_110kV_CN_269748077_110000_CN_269748078_110000/RConn2
  Te_Apiti_Woodville_110kV_CN_269748077_110000_CN_269748078_110000/RConn3 -- T_269748078_110000_Te_Apiti_substation/LConn3 -- bus67/LConn1
  T_93707134__/LConn1 -- _CN_93707134_110000_CN_270022030_110000/RConn1
  T_93707134__/LConn2 -- _CN_93707134_110000_CN_270022030_110000/RConn2
  _CN_93707134_110000_CN_270022030_110000/RConn3 -- T_93707134__/LConn3 -- bus68/LConn1
  Otahuhu_Penrose_110kV_CN_87495237_110000_CN_363290611_110000/RConn1 -- T_363290611__/LConn1 -- Mangere_Mount_Roskill_110kV;_Mount_Roskill_Otahuhu_110kV;_Mount_Roskill_Otahuhu_110kV_CN_27030962_110000_CN_363290611_110000/RConn1
  Otahuhu_Penrose_110kV_CN_87495237_110000_CN_363290611_110000/RConn2 -- T_363290611__/LConn2 -- Mangere_Mount_Roskill_110kV;_Mount_Roskill_Otahuhu_110kV;_Mount_Roskill_Otahuhu_110kV_CN_27030962_110000_CN_363290611_110000/RConn2
  Otahuhu_Penrose_110kV_CN_87495237_110000_CN_363290611_110000/RConn3 -- T_363290611__/LConn3 -- Mangere_Mount_Roskill_110kV;_Mount_Roskill_Otahuhu_110kV;_Mount_Roskill_Otahuhu_110kV_CN_27030962_110000_CN_363290611_110000/RConn3 -- bus69/LConn1
  _CN_87495237_110000_CN_359449581_110000/RConn1 -- T_359449581_220000;110000;33000;22000_Penrose_substation_(220kV)/RConn1 -- L_359449581/LConn1
  _CN_87495237_110000_CN_359449581_110000/RConn2 -- T_359449581_220000;110000;33000;22000_Penrose_substation_(220kV)/RConn2 -- L_359449581/LConn2
  _CN_87495237_110000_CN_359449581_110000/RConn3 -- T_359449581_220000;110000;33000;22000_Penrose_substation_(220kV)/RConn3 -- L_359449581/LConn3 -- bus70/LConn1
  _CN_95343088_110000_CN_34937276_110000/LConn1 -- T_95343088_110000;33000_Takapu_Road_substation/LConn1 -- Takapu_Road_Wilton_110kV_CN_95343088_110000_CN_95343089_110000/RConn1
  _CN_95343088_110000_CN_34937276_110000/LConn2 -- T_95343088_110000;33000_Takapu_Road_substation/LConn2 -- Takapu_Road_Wilton_110kV_CN_95343088_110000_CN_95343089_110000/RConn2
  _CN_95343088_110000_CN_34937276_110000/LConn3 -- T_95343088_110000;33000_Takapu_Road_substation/LConn3 -- Takapu_Road_Wilton_110kV_CN_95343088_110000_CN_95343089_110000/RConn3 -- bus71/LConn1
  T_34937276_110000;33000_Pauatahanui_substation/LConn1 -- _CN_95343088_110000_CN_34937276_110000/RConn1
  T_34937276_110000;33000_Pauatahanui_substation/LConn2 -- _CN_95343088_110000_CN_34937276_110000/RConn2
  _CN_95343088_110000_CN_34937276_110000/RConn3 -- T_34937276_110000;33000_Pauatahanui_substation/LConn3 -- bus72/LConn1
  T_193039355_110000_Mangaturoto_substation/LConn1 -- _CN_168228811_110000_CN_193039355_110000/RConn1
  T_193039355_110000_Mangaturoto_substation/LConn2 -- _CN_168228811_110000_CN_193039355_110000/RConn2
  _CN_168228811_110000_CN_193039355_110000/RConn3 -- T_193039355_110000_Mangaturoto_substation/LConn3 -- bus73/LConn1
  Bromley_Islington_220kV_CN_100957314_220000_CN_33795353_220000/LConn1 -- T_100957314_220000;66000_Bromley_substation/LConn1 -- Bromley_Islington_220kV_CN_100957314_220000_CN_268826084_220000/LConn1
  Bromley_Islington_220kV_CN_100957314_220000_CN_33795353_220000/LConn2 -- T_100957314_220000;66000_Bromley_substation/LConn2 -- Bromley_Islington_220kV_CN_100957314_220000_CN_268826084_220000/LConn2
  Bromley_Islington_220kV_CN_100957314_220000_CN_33795353_220000/LConn3 -- T_100957314_220000;66000_Bromley_substation/LConn3 -- Bromley_Islington_220kV_CN_100957314_220000_CN_268826084_220000/LConn3 -- bus74/LConn1
  Bromley_Islington_220kV_CN_100957314_220000_CN_33795353_220000/RConn1 -- T_33795353_220000;66000;33000_Islington_substation/LConn1 -- Benmore_Islington_220kV_CN_33795353_220000_CN_89664063_220000/LConn1 -- Islington_Roxburgh_220kV_CN_33795353_220000_CN_94840399_220000/LConn1
  Bromley_Islington_220kV_CN_100957314_220000_CN_33795353_220000/RConn2 -- T_33795353_220000;66000;33000_Islington_substation/LConn2 -- Benmore_Islington_220kV_CN_33795353_220000_CN_89664063_220000/LConn2 -- Islington_Roxburgh_220kV_CN_33795353_220000_CN_94840399_220000/LConn2
  Bromley_Islington_220kV_CN_100957314_220000_CN_33795353_220000/RConn3 -- T_33795353_220000;66000;33000_Islington_substation/LConn3 -- Benmore_Islington_220kV_CN_33795353_220000_CN_89664063_220000/LConn3 -- Islington_Roxburgh_220kV_CN_33795353_220000_CN_94840399_220000/LConn3 -- bus75/LConn1
  T_268826084_220000;66000;33000_Ashburton_substation/LConn1 -- Bromley_Islington_220kV_CN_100957314_220000_CN_268826084_220000/RConn1
  T_268826084_220000;66000;33000_Ashburton_substation/LConn2 -- Bromley_Islington_220kV_CN_100957314_220000_CN_268826084_220000/RConn2
  Bromley_Islington_220kV_CN_100957314_220000_CN_268826084_220000/RConn3 -- T_268826084_220000;66000;33000_Ashburton_substation/LConn3 -- bus76/LConn1
  T_329266069__/LConn1 -- _CN_329266069_220000_CN_75609279_220000/LConn1
  T_329266069__/LConn2 -- _CN_329266069_220000_CN_75609279_220000/LConn2
  _CN_329266069_220000_CN_75609279_220000/LConn3 -- T_329266069__/LConn3 -- bus77/LConn1
  _CN_329266069_220000_CN_75609279_220000/RConn1 -- T_75609279_220000;110000_Otahuhu_substation/LConn1 -- _CN_329266072_220000_CN_75609279_220000/LConn1 -- Henderson_Otahuhu_220kV_CN_87897292_220000_CN_75609279_220000/LConn1 -- Otahuhu_Whakamaru_B_CN_87837416_220000_CN_75609279_220000/LConn1
  _CN_329266069_220000_CN_75609279_220000/RConn2 -- T_75609279_220000;110000_Otahuhu_substation/LConn2 -- _CN_329266072_220000_CN_75609279_220000/LConn2 -- Henderson_Otahuhu_220kV_CN_87897292_220000_CN_75609279_220000/LConn2 -- Otahuhu_Whakamaru_B_CN_87837416_220000_CN_75609279_220000/LConn2
  _CN_329266069_220000_CN_75609279_220000/RConn3 -- T_75609279_220000;110000_Otahuhu_substation/LConn3 -- _CN_329266072_220000_CN_75609279_220000/LConn3 -- Henderson_Otahuhu_220kV_CN_87897292_220000_CN_75609279_220000/LConn3 -- Otahuhu_Whakamaru_B_CN_87837416_220000_CN_75609279_220000/LConn3 -- bus78/LConn1
  T_180514007_220000;110000_Roxburgh_substation/LConn1 -- Islington_Roxburgh_220kV_CN_180514007_220000_CN_414953388_220000/LConn1
  T_180514007_220000;110000_Roxburgh_substation/LConn2 -- Islington_Roxburgh_220kV_CN_180514007_220000_CN_414953388_220000/LConn2
  Islington_Roxburgh_220kV_CN_180514007_220000_CN_414953388_220000/LConn3 -- T_180514007_220000;110000_Roxburgh_substation/LConn3 -- bus79/LConn1
  Islington_Roxburgh_220kV_CN_180514007_220000_CN_414953388_220000/RConn1 -- T_414953388_220000;33000_Naesby_substation/LConn1 -- Islington_Roxburgh_220kV_CN_414953388_220000_CN_94840399_220000/LConn1
  Islington_Roxburgh_220kV_CN_180514007_220000_CN_414953388_220000/RConn2 -- T_414953388_220000;33000_Naesby_substation/LConn2 -- Islington_Roxburgh_220kV_CN_414953388_220000_CN_94840399_220000/LConn2
  Islington_Roxburgh_220kV_CN_180514007_220000_CN_414953388_220000/RConn3 -- T_414953388_220000;33000_Naesby_substation/LConn3 -- Islington_Roxburgh_220kV_CN_414953388_220000_CN_94840399_220000/LConn3 -- bus80/LConn1
  T_26671244_220000;110000;33000_Henderson_substation/LConn1 -- _CN_26671244_220000_CN_232382576_220000/LConn1
  T_26671244_220000;110000;33000_Henderson_substation/LConn2 -- _CN_26671244_220000_CN_232382576_220000/LConn2
  _CN_26671244_220000_CN_232382576_220000/LConn3 -- T_26671244_220000;110000;33000_Henderson_substation/LConn3 -- bus81/LConn1
  T_232382576_220000;110000_Marsden_substation/LConn1 -- _CN_26671244_220000_CN_232382576_220000/RConn1
  T_232382576_220000;110000_Marsden_substation/LConn2 -- _CN_26671244_220000_CN_232382576_220000/RConn2
  _CN_26671244_220000_CN_232382576_220000/RConn3 -- T_232382576_220000;110000_Marsden_substation/LConn3 -- bus82/LConn1
  T_161270797_220000;110000;33000_Albany_substation/LConn1 -- _CN_161270797_220000_CN_95894638_220000/LConn1
  T_161270797_220000;110000;33000_Albany_substation/LConn2 -- _CN_161270797_220000_CN_95894638_220000/LConn2
  _CN_161270797_220000_CN_95894638_220000/LConn3 -- T_161270797_220000;110000;33000_Albany_substation/LConn3 -- bus83/LConn1
  _CN_161270797_220000_CN_95894638_220000/RConn1 -- T_95894638_220000;110000;33000_Wairau_Road_substation/LConn1 -- _CN_95894638_220000_CN_156097401_220000/LConn1
  _CN_161270797_220000_CN_95894638_220000/RConn2 -- T_95894638_220000;110000;33000_Wairau_Road_substation/LConn2 -- _CN_95894638_220000_CN_156097401_220000/LConn2
  _CN_161270797_220000_CN_95894638_220000/RConn3 -- T_95894638_220000;110000;33000_Wairau_Road_substation/LConn3 -- _CN_95894638_220000_CN_156097401_220000/LConn3 -- bus84/LConn1
  T_270556206_220000_Ohaaki_substation/LConn1 -- _CN_270556206_220000_CN_143397051_220000/LConn1
  T_270556206_220000_Ohaaki_substation/LConn2 -- _CN_270556206_220000_CN_143397051_220000/LConn2
  _CN_270556206_220000_CN_143397051_220000/LConn3 -- T_270556206_220000_Ohaaki_substation/LConn3 -- bus85/LConn1
  G_143397051_Ohaaki_Power_Station/RConn1 -- _CN_270556206_220000_CN_143397051_220000/RConn1
  G_143397051_Ohaaki_Power_Station/RConn2 -- _CN_270556206_220000_CN_143397051_220000/RConn2
  _CN_270556206_220000_CN_143397051_220000/RConn3 -- G_143397051_Ohaaki_Power_Station/RConn3 -- bus86/LConn1
  T_329266072__/LConn1 -- _CN_329266072_220000_CN_75609279_220000/RConn1
  T_329266072__/LConn2 -- _CN_329266072_220000_CN_75609279_220000/RConn2
  _CN_329266072_220000_CN_75609279_220000/RConn3 -- T_329266072__/LConn3 -- bus87/LConn1
  T_270018358_220000_Aratiatia_substation/LConn1 -- _CN_270018358_220000_CN_410732354_220000/LConn1
  T_270018358_220000_Aratiatia_substation/LConn2 -- _CN_270018358_220000_CN_410732354_220000/LConn2
  _CN_270018358_220000_CN_410732354_220000/LConn3 -- T_270018358_220000_Aratiatia_substation/LConn3 -- bus88/LConn1
  G_410732354_Aratiatia_power_station/RConn1 -- _CN_270018358_220000_CN_410732354_220000/RConn1
  G_410732354_Aratiatia_power_station/RConn2 -- _CN_270018358_220000_CN_410732354_220000/RConn2
  _CN_270018358_220000_CN_410732354_220000/RConn3 -- G_410732354_Aratiatia_power_station/RConn3 -- bus89/LConn1
  T_255873374_220000_Ngatamariki_substation/LConn1 -- _CN_255873374_220000_CN_270554679_220000/LConn1
  T_255873374_220000_Ngatamariki_substation/LConn2 -- _CN_255873374_220000_CN_270554679_220000/LConn2
  _CN_255873374_220000_CN_270554679_220000/LConn3 -- T_255873374_220000_Ngatamariki_substation/LConn3 -- bus90/LConn1
  T_270554679_220000_Nga_Awa_Purua_substation/LConn1 -- _CN_255873374_220000_CN_270554679_220000/RConn1
  T_270554679_220000_Nga_Awa_Purua_substation/LConn2 -- _CN_255873374_220000_CN_270554679_220000/RConn2
  _CN_255873374_220000_CN_270554679_220000/RConn3 -- T_270554679_220000_Nga_Awa_Purua_substation/LConn3 -- bus91/LConn1
  Benmore_Islington_220kV_CN_33795353_220000_CN_89664063_220000/RConn1 -- T_89664063_220000_Benmore_(HVAC)_substation/LConn1 -- _CN_89664057_220000_CN_89664063_220000/LConn1 -- _CN_89664063_220000_CN_89665166_220000/LConn1 -- Benmore_Twizel_220kV_CN_89664063_220000_CN_89635947_220000/LConn1
  Benmore_Islington_220kV_CN_33795353_220000_CN_89664063_220000/RConn2 -- T_89664063_220000_Benmore_(HVAC)_substation/LConn2 -- _CN_89664057_220000_CN_89664063_220000/LConn2 -- _CN_89664063_220000_CN_89665166_220000/LConn2 -- Benmore_Twizel_220kV_CN_89664063_220000_CN_89635947_220000/LConn2
  Benmore_Islington_220kV_CN_33795353_220000_CN_89664063_220000/RConn3 -- T_89664063_220000_Benmore_(HVAC)_substation/LConn3 -- _CN_89664057_220000_CN_89664063_220000/LConn3 -- _CN_89664063_220000_CN_89665166_220000/LConn3 -- Benmore_Twizel_220kV_CN_89664063_220000_CN_89635947_220000/LConn3 -- bus92/LConn1
  Islington_Roxburgh_220kV_CN_33795353_220000_CN_94840399_220000/RConn1 -- T_94840399_220000_Livingstone_switching_station/LConn1 -- Islington_Roxburgh_220kV_CN_414953388_220000_CN_94840399_220000/RConn1 -- _CN_89637173_220000_CN_94840399_220000/LConn1
  Islington_Roxburgh_220kV_CN_33795353_220000_CN_94840399_220000/RConn2 -- T_94840399_220000_Livingstone_switching_station/LConn2 -- Islington_Roxburgh_220kV_CN_414953388_220000_CN_94840399_220000/RConn2 -- _CN_89637173_220000_CN_94840399_220000/LConn2
  Islington_Roxburgh_220kV_CN_33795353_220000_CN_94840399_220000/RConn3 -- T_94840399_220000_Livingstone_switching_station/LConn3 -- Islington_Roxburgh_220kV_CN_414953388_220000_CN_94840399_220000/RConn3 -- _CN_89637173_220000_CN_94840399_220000/LConn3 -- bus93/LConn1
  T_89636510_220000_Ohau_A_substation/LConn1 -- Ohau_A_Twizel_220kV_CN_89636510_220000_CN_170300247_220000/LConn1
  T_89636510_220000_Ohau_A_substation/LConn2 -- Ohau_A_Twizel_220kV_CN_89636510_220000_CN_170300247_220000/LConn2
  Ohau_A_Twizel_220kV_CN_89636510_220000_CN_170300247_220000/LConn3 -- T_89636510_220000_Ohau_A_substation/LConn3 -- bus94/LConn1
  T_170300247_220000;33000_Twizel_substation/LConn1 -- Ohau_A_Twizel_220kV_CN_89636510_220000_CN_170300247_220000/RConn1
  T_170300247_220000;33000_Twizel_substation/LConn2 -- Ohau_A_Twizel_220kV_CN_89636510_220000_CN_170300247_220000/RConn2
  Ohau_A_Twizel_220kV_CN_89636510_220000_CN_170300247_220000/RConn3 -- T_170300247_220000;33000_Twizel_substation/LConn3 -- bus95/LConn1
  T_89636266_220000_Ohau_C_substation/LConn1 -- _CN_89636266_220000_CN_165279371_220000/LConn1
  T_89636266_220000_Ohau_C_substation/LConn2 -- _CN_89636266_220000_CN_165279371_220000/LConn2
  _CN_89636266_220000_CN_165279371_220000/LConn3 -- T_89636266_220000_Ohau_C_substation/LConn3 -- bus96/LConn1
  G_165279371_Ohau_C_powerhouse/RConn1 -- _CN_89636266_220000_CN_165279371_220000/RConn1
  G_165279371_Ohau_C_powerhouse/RConn2 -- _CN_89636266_220000_CN_165279371_220000/RConn2
  _CN_89636266_220000_CN_165279371_220000/RConn3 -- G_165279371_Ohau_C_powerhouse/RConn3 -- bus97/LConn1
  _CN_89411122_220000_CN_87837416_220000/LConn1 -- T_89411122_220000;33000_Tokaanu_substation/LConn1 -- _CN_89411122_220000_CN_167285336_220000/LConn1
  _CN_89411122_220000_CN_87837416_220000/LConn2 -- T_89411122_220000;33000_Tokaanu_substation/LConn2 -- _CN_89411122_220000_CN_167285336_220000/LConn2
  _CN_89411122_220000_CN_87837416_220000/LConn3 -- T_89411122_220000;33000_Tokaanu_substation/LConn3 -- _CN_89411122_220000_CN_167285336_220000/LConn3 -- bus98/LConn1
  _CN_89411122_220000_CN_87837416_220000/RConn1 -- T_87837416_220000_Whakamaru_substation/LConn1 -- _CN_87837416_220000_CN_409970312_220000/LConn1 -- Wairakei_Whakamaru_220kV_line_A_CN_87837416_220000_CN_272522517_220000/LConn1 -- Maraetai_Whakamaru_220kV_line_B_CN_270550888_220000_CN_87837416_220000/LConn1 -- Otahuhu_Whakamaru_B_CN_87837416_220000_CN_75609279_220000/RConn1
  _CN_89411122_220000_CN_87837416_220000/RConn2 -- T_87837416_220000_Whakamaru_substation/LConn2 -- _CN_87837416_220000_CN_409970312_220000/LConn2 -- Wairakei_Whakamaru_220kV_line_A_CN_87837416_220000_CN_272522517_220000/LConn2 -- Maraetai_Whakamaru_220kV_line_B_CN_270550888_220000_CN_87837416_220000/LConn2 -- Otahuhu_Whakamaru_B_CN_87837416_220000_CN_75609279_220000/RConn2
  _CN_89411122_220000_CN_87837416_220000/RConn3 -- T_87837416_220000_Whakamaru_substation/LConn3 -- _CN_87837416_220000_CN_409970312_220000/LConn3 -- Wairakei_Whakamaru_220kV_line_A_CN_87837416_220000_CN_272522517_220000/LConn3 -- bus99/LConn1 -- Maraetai_Whakamaru_220kV_line_B_CN_270550888_220000_CN_87837416_220000/LConn3 -- Otahuhu_Whakamaru_B_CN_87837416_220000_CN_75609279_220000/RConn3
  _CN_89411122_220000_CN_167285336_220000/RConn1 -- T_167285336_220000;110000;50000;33000_Bunnythorpe_substation/LConn1 -- Bunnythorpe_Wairakei_220kV_CN_167285260_220000_CN_167285336_220000/LConn1 -- Bunnythorpe_Haywards_220kV_line_B_CN_167285336_220000_CN_93713118_220000/LConn1
  _CN_89411122_220000_CN_167285336_220000/RConn2 -- T_167285336_220000;110000;50000;33000_Bunnythorpe_substation/LConn2 -- Bunnythorpe_Wairakei_220kV_CN_167285260_220000_CN_167285336_220000/LConn2 -- Bunnythorpe_Haywards_220kV_line_B_CN_167285336_220000_CN_93713118_220000/LConn2
  _CN_89411122_220000_CN_167285336_220000/RConn3 -- T_167285336_220000;110000;50000;33000_Bunnythorpe_substation/LConn3 -- Bunnythorpe_Wairakei_220kV_CN_167285260_220000_CN_167285336_220000/LConn3 -- Bunnythorpe_Haywards_220kV_line_B_CN_167285336_220000_CN_93713118_220000/LConn3 -- bus100/LConn1
  _CN_89637173_220000_CN_89637174_220000/LConn1 -- T_89637173_220000;110000;33000;11000_Waitaki_substation/LConn1 -- _CN_89637173_220000_CN_94840399_220000/RConn1
  _CN_89637173_220000_CN_89637174_220000/LConn2 -- T_89637173_220000;110000;33000;11000_Waitaki_substation/LConn2 -- _CN_89637173_220000_CN_94840399_220000/RConn2
  _CN_89637173_220000_CN_89637174_220000/LConn3 -- T_89637173_220000;110000;33000;11000_Waitaki_substation/LConn3 -- _CN_89637173_220000_CN_94840399_220000/RConn3 -- bus101/LConn1
  T_89637174_220000_Aviemore_substation/LConn1 -- _CN_89637173_220000_CN_89637174_220000/RConn1
  T_89637174_220000_Aviemore_substation/LConn2 -- _CN_89637173_220000_CN_89637174_220000/RConn2
  _CN_89637173_220000_CN_89637174_220000/RConn3 -- T_89637174_220000_Aviemore_substation/LConn3 -- bus102/LConn1
  T_89664057_350000;220000_Benmore_HVDC_static_inverter_station/LConn1 -- _CN_89664057_220000_CN_89664063_220000/RConn1
  T_89664057_350000;220000_Benmore_HVDC_static_inverter_station/LConn2 -- _CN_89664057_220000_CN_89664063_220000/RConn2
  _CN_89664057_220000_CN_89664063_220000/RConn3 -- T_89664057_350000;220000_Benmore_HVDC_static_inverter_station/LConn3 -- bus103/LConn1
  G_89665166_Benmore/RConn1 -- _CN_89664063_220000_CN_89665166_220000/RConn1
  G_89665166_Benmore/RConn2 -- _CN_89664063_220000_CN_89665166_220000/RConn2
  _CN_89664063_220000_CN_89665166_220000/RConn3 -- G_89665166_Benmore/RConn3 -- bus104/LConn1
  T_89635947_220000_Ohau_B_substation/LConn1 -- Benmore_Twizel_220kV_CN_89664063_220000_CN_89635947_220000/RConn1
  T_89635947_220000_Ohau_B_substation/LConn2 -- Benmore_Twizel_220kV_CN_89664063_220000_CN_89635947_220000/RConn2
  Benmore_Twizel_220kV_CN_89664063_220000_CN_89635947_220000/RConn3 -- T_89635947_220000_Ohau_B_substation/LConn3 -- bus105/LConn1
  T_270550888__Maraetai_I_substation/LConn1 -- Maraetai_Whakamaru_220kV_line_B_CN_270550888_220000_CN_87837416_220000/RConn1
  T_270550888__Maraetai_I_substation/LConn2 -- Maraetai_Whakamaru_220kV_line_B_CN_270550888_220000_CN_87837416_220000/RConn2
  Maraetai_Whakamaru_220kV_line_B_CN_270550888_220000_CN_87837416_220000/RConn3 -- T_270550888__Maraetai_I_substation/LConn3 -- bus106/LConn1
  T_167285260_220000;33000_Wairakei_substation/LConn1 -- Bunnythorpe_Wairakei_220kV_CN_167285260_220000_CN_167285336_220000/RConn1
  T_167285260_220000;33000_Wairakei_substation/LConn2 -- Bunnythorpe_Wairakei_220kV_CN_167285260_220000_CN_167285336_220000/RConn2
  Bunnythorpe_Wairakei_220kV_CN_167285260_220000_CN_167285336_220000/RConn3 -- T_167285260_220000;33000_Wairakei_substation/LConn3 -- bus107/LConn1
  T_412588974_220000_Tiwai_substation/LConn1 -- _CN_412588974_220000_CN_268841395_220000/LConn1
  T_412588974_220000_Tiwai_substation/LConn2 -- _CN_412588974_220000_CN_268841395_220000/LConn2
  _CN_412588974_220000_CN_268841395_220000/LConn3 -- T_412588974_220000_Tiwai_substation/LConn3 -- bus108/LConn1
  T_268841395_220000_North_Makarewa_substation/LConn1 -- _CN_412588974_220000_CN_268841395_220000/RConn1
  T_268841395_220000_North_Makarewa_substation/LConn2 -- _CN_412588974_220000_CN_268841395_220000/RConn2
  _CN_412588974_220000_CN_268841395_220000/RConn3 -- T_268841395_220000_North_Makarewa_substation/LConn3 -- bus109/LConn1
  T_87897292_220000_Southdown_substation/LConn1 -- Henderson_Otahuhu_220kV_CN_87897292_220000_CN_75609279_220000/RConn1
  T_87897292_220000_Southdown_substation/LConn2 -- Henderson_Otahuhu_220kV_CN_87897292_220000_CN_75609279_220000/RConn2
  Henderson_Otahuhu_220kV_CN_87897292_220000_CN_75609279_220000/RConn3 -- T_87897292_220000_Southdown_substation/LConn3 -- bus110/LConn1
  T_169512273__/LConn1 -- _CN_169512273_220000_CN_87928925_220000/LConn1
  T_169512273__/LConn2 -- _CN_169512273_220000_CN_87928925_220000/LConn2
  _CN_169512273_220000_CN_87928925_220000/LConn3 -- T_169512273__/LConn3 -- bus111/LConn1
  T_87928925__Maraetai_II_sub_station/LConn1 -- _CN_169512273_220000_CN_87928925_220000/RConn1
  T_87928925__Maraetai_II_sub_station/LConn2 -- _CN_169512273_220000_CN_87928925_220000/RConn2
  _CN_169512273_220000_CN_87928925_220000/RConn3 -- T_87928925__Maraetai_II_sub_station/LConn3 -- bus112/LConn1
  _CN_341099346_220000_CN_156094589_220000/LConn1 -- T_341099346__Pakuranga_substation_(new)/LConn1 -- _CN_341099346_220000_CN_359449581_220000/LConn1
  _CN_341099346_220000_CN_156094589_220000/LConn2 -- T_341099346__Pakuranga_substation_(new)/LConn2 -- _CN_341099346_220000_CN_359449581_220000/LConn2
  _CN_341099346_220000_CN_156094589_220000/LConn3 -- T_341099346__Pakuranga_substation_(new)/LConn3 -- _CN_341099346_220000_CN_359449581_220000/LConn3 -- bus113/LConn1
  T_156094589_220000_Brownhill_substation/LConn1 -- _CN_341099346_220000_CN_156094589_220000/RConn1
  T_156094589_220000_Brownhill_substation/LConn2 -- _CN_341099346_220000_CN_156094589_220000/RConn2
  _CN_341099346_220000_CN_156094589_220000/RConn3 -- T_156094589_220000_Brownhill_substation/LConn3 -- bus114/LConn1
  _CN_341099346_220000_CN_359449581_220000/RConn1 -- T_359449581_220000;110000;33000;22000_Penrose_substation_(220kV)/LConn1 -- _CN_359449581_220000_CN_156097401_220000/LConn1
  _CN_341099346_220000_CN_359449581_220000/RConn2 -- T_359449581_220000;110000;33000;22000_Penrose_substation_(220kV)/LConn2 -- _CN_359449581_220000_CN_156097401_220000/LConn2
  _CN_341099346_220000_CN_359449581_220000/RConn3 -- T_359449581_220000;110000;33000;22000_Penrose_substation_(220kV)/LConn3 -- _CN_359449581_220000_CN_156097401_220000/LConn3 -- bus115/LConn1
  T_270022030_220000;110000;11000_Tarukenga_substation/LConn1 -- Edgecumbe_Tarukenga_220kV_CN_270022030_220000_CN_167283894_220000/LConn1
  T_270022030_220000;110000;11000_Tarukenga_substation/LConn2 -- Edgecumbe_Tarukenga_220kV_CN_270022030_220000_CN_167283894_220000/LConn2
  Edgecumbe_Tarukenga_220kV_CN_270022030_220000_CN_167283894_220000/LConn3 -- T_270022030_220000;110000;11000_Tarukenga_substation/LConn3 -- bus116/LConn1
  Edgecumbe_Tarukenga_220kV_CN_270022030_220000_CN_167283894_220000/RConn1 -- T_167283894_220000;110000;33000_Edgecumbe_substation/LConn1 -- Edgecumbe_Ohakuri_220kV_CN_167283894_220000_CN_272522517_220000/LConn1
  Edgecumbe_Tarukenga_220kV_CN_270022030_220000_CN_167283894_220000/RConn2 -- T_167283894_220000;110000;33000_Edgecumbe_substation/LConn2 -- Edgecumbe_Ohakuri_220kV_CN_167283894_220000_CN_272522517_220000/LConn2
  Edgecumbe_Tarukenga_220kV_CN_270022030_220000_CN_167283894_220000/RConn3 -- T_167283894_220000;110000;33000_Edgecumbe_substation/LConn3 -- Edgecumbe_Ohakuri_220kV_CN_167283894_220000_CN_272522517_220000/LConn3 -- bus117/LConn1
  Bunnythorpe_Haywards_220kV_line_B_CN_167285336_220000_CN_93713118_220000/RConn1 -- T_93713118_220000;110000;33000;11000_Haywards_substation/LConn1 -- _CN_93713115_220000_CN_93713118_220000/LConn1
  Bunnythorpe_Haywards_220kV_line_B_CN_167285336_220000_CN_93713118_220000/RConn2 -- T_93713118_220000;110000;33000;11000_Haywards_substation/LConn2 -- _CN_93713115_220000_CN_93713118_220000/LConn2
  Bunnythorpe_Haywards_220kV_line_B_CN_167285336_220000_CN_93713118_220000/RConn3 -- T_93713118_220000;110000;33000;11000_Haywards_substation/LConn3 -- _CN_93713115_220000_CN_93713118_220000/LConn3 -- bus118/LConn1
  T_93713115_350000;220000_Haywards_static_inverter_plant/LConn1 -- _CN_93713115_220000_CN_93713118_220000/RConn1
  T_93713115_350000;220000_Haywards_static_inverter_plant/LConn2 -- _CN_93713115_220000_CN_93713118_220000/RConn2
  _CN_93713115_220000_CN_93713118_220000/RConn3 -- T_93713115_350000;220000_Haywards_static_inverter_plant/LConn3 -- bus119/LConn1
  Edgecumbe_Ohakuri_220kV_CN_167283894_220000_CN_272522517_220000/RConn1 -- T_272522517_220000_Ohakuri_substation/LConn1 -- Wairakei_Whakamaru_220kV_line_A_CN_87837416_220000_CN_272522517_220000/RConn1
  Edgecumbe_Ohakuri_220kV_CN_167283894_220000_CN_272522517_220000/RConn2 -- T_272522517_220000_Ohakuri_substation/LConn2 -- Wairakei_Whakamaru_220kV_line_A_CN_87837416_220000_CN_272522517_220000/RConn2
  Edgecumbe_Ohakuri_220kV_CN_167283894_220000_CN_272522517_220000/RConn3 -- T_272522517_220000_Ohakuri_substation/LConn3 -- Wairakei_Whakamaru_220kV_line_A_CN_87837416_220000_CN_272522517_220000/RConn3 -- bus120/LConn1
  G_409970312_Whakamaru_power_station/RConn1 -- _CN_87837416_220000_CN_409970312_220000/RConn1
  G_409970312_Whakamaru_power_station/RConn2 -- _CN_87837416_220000_CN_409970312_220000/RConn2
  _CN_87837416_220000_CN_409970312_220000/RConn3 -- G_409970312_Whakamaru_power_station/RConn3 -- bus121/LConn1
  T_270012796_220000_Tekapo_B_substation/LConn1 -- _CN_270012796_220000_CN_270012792_220000/LConn1
  T_270012796_220000_Tekapo_B_substation/LConn2 -- _CN_270012796_220000_CN_270012792_220000/LConn2
  _CN_270012796_220000_CN_270012792_220000/LConn3 -- T_270012796_220000_Tekapo_B_substation/LConn3 -- bus122/LConn1
  G_270012792_Tekapo_B/RConn1 -- _CN_270012796_220000_CN_270012792_220000/RConn1
  G_270012792_Tekapo_B/RConn2 -- _CN_270012796_220000_CN_270012792_220000/RConn2
  _CN_270012796_220000_CN_270012792_220000/RConn3 -- G_270012792_Tekapo_B/RConn3 -- bus123/LConn1
  _CN_359449581_220000_CN_156097401_220000/RConn1 -- T_156097401_220000;110000;22000;11000_Hobson_Street_substation/LConn1 -- _CN_95894638_220000_CN_156097401_220000/RConn1
  _CN_359449581_220000_CN_156097401_220000/RConn2 -- T_156097401_220000;110000;22000;11000_Hobson_Street_substation/LConn2 -- _CN_95894638_220000_CN_156097401_220000/RConn2
  _CN_359449581_220000_CN_156097401_220000/RConn3 -- T_156097401_220000;110000;22000;11000_Hobson_Street_substation/LConn3 -- _CN_95894638_220000_CN_156097401_220000/RConn3 -- bus124/LConn1
  T_412589726_220000_Manapouri_substation/LConn1 -- _CN_412589726_220000_CN_194912653_220000/LConn1
  T_412589726_220000_Manapouri_substation/LConn2 -- _CN_412589726_220000_CN_194912653_220000/LConn2
  _CN_412589726_220000_CN_194912653_220000/LConn3 -- T_412589726_220000_Manapouri_substation/LConn3 -- bus125/LConn1
  G_194912653_Manapouri_Power_Station/RConn1 -- _CN_412589726_220000_CN_194912653_220000/RConn1
  G_194912653_Manapouri_Power_Station/RConn2 -- _CN_412589726_220000_CN_194912653_220000/RConn2
  _CN_412589726_220000_CN_194912653_220000/RConn3 -- G_194912653_Manapouri_Power_Station/RConn3 -- bus126/LConn1
  T_400732687__/RConn1 -- L_400732687/LConn1
  T_400732687__/RConn2 -- L_400732687/LConn2
  L_400732687/LConn3 -- T_400732687__/RConn3 -- bus127/LConn1
  T_173729963_110000;50000_Gisborne_substation/RConn1 -- L_173729963/LConn1
  T_173729963_110000;50000_Gisborne_substation/RConn2 -- L_173729963/LConn2
  L_173729963/LConn3 -- T_173729963_110000;50000_Gisborne_substation/RConn3 -- bus128/LConn1
  T_167434770_110000;11000_Te_Awamutu_substation/RConn1 -- L_167434770/LConn1
  T_167434770_110000;11000_Te_Awamutu_substation/RConn2 -- L_167434770/LConn2
  L_167434770/LConn3 -- T_167434770_110000;11000_Te_Awamutu_substation/RConn3 -- bus129/LConn1
  T_270536018_110000_Karapiro_substation/RConn1 -- L_270536018/LConn1
  T_270536018_110000_Karapiro_substation/RConn2 -- L_270536018/LConn2
  L_270536018/LConn3 -- T_270536018_110000_Karapiro_substation/RConn3 -- bus130/LConn1
  T_167425043_110000;11000_Ohakune_substation/RConn1 -- L_167425043/LConn1
  T_167425043_110000;11000_Ohakune_substation/RConn2 -- L_167425043/LConn2
  L_167425043/LConn3 -- T_167425043_110000;11000_Ohakune_substation/RConn3 -- bus131/LConn1
  T_410151576_110000;33000_Ongarue_substation/RConn1 -- L_410151576/LConn1
  T_410151576_110000;33000_Ongarue_substation/RConn2 -- L_410151576/LConn2
  L_410151576/LConn3 -- T_410151576_110000;33000_Ongarue_substation/RConn3 -- bus132/LConn1
  T_367205270_110000;33000_Mataroa_substation/RConn1 -- L_367205270/LConn1
  T_367205270_110000;33000_Mataroa_substation/RConn2 -- L_367205270/LConn2
  L_367205270/LConn3 -- T_367205270_110000;33000_Mataroa_substation/RConn3 -- bus133/LConn1
  T_168951331__Wheao_substation/RConn1 -- L_168951331/LConn1
  T_168951331__Wheao_substation/RConn2 -- L_168951331/LConn2
  L_168951331/LConn3 -- T_168951331__Wheao_substation/RConn3 -- bus134/LConn1
  T_93844343_110000;33000;11000_Rotorua_substation/RConn1 -- L_93844343/LConn1
  T_93844343_110000;33000;11000_Rotorua_substation/RConn2 -- L_93844343/LConn2
  L_93844343/LConn3 -- T_93844343_110000;33000;11000_Rotorua_substation/RConn3 -- bus135/LConn1
  T_232293420_110000_Tuai_substation/RConn1 -- L_232293420/LConn1
  T_232293420_110000_Tuai_substation/RConn2 -- L_232293420/LConn2
  L_232293420/LConn3 -- T_232293420_110000_Tuai_substation/RConn3 -- bus136/LConn1
  T_413551915_110000;50000;33000;11000_Wairoa_substation/RConn1 -- L_413551915/LConn1
  T_413551915_110000;50000;33000;11000_Wairoa_substation/RConn2 -- L_413551915/LConn2
  L_413551915/LConn3 -- T_413551915_110000;50000;33000;11000_Wairoa_substation/RConn3 -- bus137/LConn1
  T_93419961_110000;33000_Fernhill_substation/RConn1 -- L_93419961/LConn1
  T_93419961_110000;33000_Fernhill_substation/RConn2 -- L_93419961/LConn2
  L_93419961/LConn3 -- T_93419961_110000;33000_Fernhill_substation/RConn3 -- bus138/LConn1
  T_187865148_110000;33000_Hangatiki_substation/RConn1 -- L_187865148/LConn1
  T_187865148_110000;33000_Hangatiki_substation/RConn2 -- L_187865148/LConn2
  L_187865148/LConn3 -- T_187865148_110000;33000_Hangatiki_substation/RConn3 -- bus139/LConn1
  T_272523195_110000_Arapuni_substation/RConn1 -- L_272523195/LConn1
  T_272523195_110000_Arapuni_substation/RConn2 -- L_272523195/LConn2
  L_272523195/LConn3 -- T_272523195_110000_Arapuni_substation/RConn3 -- bus140/LConn1
  T_168231493_110000_Inangahua_substation/RConn1 -- L_168231493/LConn1
  T_168231493_110000_Inangahua_substation/RConn2 -- L_168231493/LConn2
  L_168231493/LConn3 -- T_168231493_110000_Inangahua_substation/RConn3 -- bus141/LConn1
  T_231527208__/RConn1 -- L_231527208/LConn1
  T_231527208__/RConn2 -- L_231527208/LConn2
  L_231527208/LConn3 -- T_231527208__/RConn3 -- bus142/LConn1
  T_90092619_110000;33000_Edendale_substation/RConn1 -- L_90092619/LConn1
  T_90092619_110000;33000_Edendale_substation/RConn2 -- L_90092619/LConn2
  L_90092619/LConn3 -- T_90092619_110000;33000_Edendale_substation/RConn3 -- bus143/LConn1
  T_224937549_110000_Brydone_substation/RConn1 -- L_224937549/LConn1
  T_224937549_110000_Brydone_substation/RConn2 -- L_224937549/LConn2
  L_224937549/LConn3 -- T_224937549_110000_Brydone_substation/RConn3 -- bus144/LConn1
  T_87338082_110000_Lichfield_substation/RConn1 -- L_87338082/LConn1
  T_87338082_110000_Lichfield_substation/RConn2 -- L_87338082/LConn2
  L_87338082/LConn3 -- T_87338082_110000_Lichfield_substation/RConn3 -- bus145/LConn1
  T_140103942__/RConn1 -- L_140103942/LConn1
  T_140103942__/RConn2 -- L_140103942/LConn2
  L_140103942/LConn3 -- T_140103942__/RConn3 -- bus146/LConn1
  T_174382184_110000;33000_Waikino_substation/RConn1 -- L_174382184/LConn1
  T_174382184_110000;33000_Waikino_substation/RConn2 -- L_174382184/LConn2
  L_174382184/LConn3 -- T_174382184_110000;33000_Waikino_substation/RConn3 -- bus147/LConn1
  T_87894783_110000;33000_Waihou_substation/RConn1 -- L_87894783/LConn1
  T_87894783_110000;33000_Waihou_substation/RConn2 -- L_87894783/LConn2
  L_87894783/LConn3 -- T_87894783_110000;33000_Waihou_substation/RConn3 -- bus148/LConn1
  T_146612611_110000;66000_Kopu_substation/RConn1 -- L_146612611/LConn1
  T_146612611_110000;66000_Kopu_substation/RConn2 -- L_146612611/LConn2
  L_146612611/LConn3 -- T_146612611_110000;66000_Kopu_substation/RConn3 -- bus149/LConn1
  T_218862188_110000;33000_Balclutha_substation/RConn1 -- L_218862188/LConn1
  T_218862188_110000;33000_Balclutha_substation/RConn2 -- L_218862188/LConn2
  L_218862188/LConn3 -- T_218862188_110000;33000_Balclutha_substation/RConn3 -- bus150/LConn1
  T_413796046_110000_Berwick_substation/RConn1 -- L_413796046/LConn1
  T_413796046_110000_Berwick_substation/RConn2 -- L_413796046/LConn2
  L_413796046/LConn3 -- T_413796046_110000_Berwick_substation/RConn3 -- bus151/LConn1
  T_51867062_110000;33000_Hepburn_Road_substation/RConn1 -- L_51867062/LConn1
  T_51867062_110000;33000_Hepburn_Road_substation/RConn2 -- L_51867062/LConn2
  L_51867062/LConn3 -- T_51867062_110000;33000_Hepburn_Road_substation/RConn3 -- bus152/LConn1
  T_168228811__Wellsford_substation/RConn1 -- L_168228811/LConn1
  T_168228811__Wellsford_substation/RConn2 -- L_168228811/LConn2
  L_168228811/LConn3 -- T_168228811__Wellsford_substation/RConn3 -- bus153/LConn1
  T_93836457_110000;33000_Huirangi_substation/RConn1 -- L_93836457/LConn1
  T_93836457_110000;33000_Huirangi_substation/RConn2 -- L_93836457/LConn2
  L_93836457/LConn3 -- T_93836457_110000;33000_Huirangi_substation/RConn3 -- bus154/LConn1
  T_93836458_110000;33000_Carrington_Street_substation/RConn1 -- L_93836458/LConn1
  T_93836458_110000;33000_Carrington_Street_substation/RConn2 -- L_93836458/LConn2
  L_93836458/LConn3 -- T_93836458_110000;33000_Carrington_Street_substation/RConn3 -- bus155/LConn1
  T_340501677_110000;11000_Cambridge_substation/RConn1 -- L_340501677/LConn1
  T_340501677_110000;11000_Cambridge_substation/RConn2 -- L_340501677/LConn2
  L_340501677/LConn3 -- T_340501677_110000;11000_Cambridge_substation/RConn3 -- bus156/LConn1
  T_94053861_220000;110000;55000;33000;11000_Hamilton_sub_station/RConn1 -- L_94053861/LConn1
  T_94053861_220000;110000;55000;33000;11000_Hamilton_sub_station/RConn2 -- L_94053861/LConn2
  L_94053861/LConn3 -- T_94053861_220000;110000;55000;33000;11000_Hamilton_sub_station/RConn3 -- bus157/LConn1
  T_93836463_220000;110000;33000_New_Plymouth_substation/RConn1 -- L_93836463/LConn1
  T_93836463_220000;110000;33000_New_Plymouth_substation/RConn2 -- L_93836463/LConn2
  L_93836463/LConn3 -- T_93836463_220000;110000;33000_New_Plymouth_substation/RConn3 -- bus158/LConn1
  T_168096434_110000;33000;11000_Waipawa_substation/RConn1 -- L_168096434/LConn1
  T_168096434_110000;33000;11000_Waipawa_substation/RConn2 -- L_168096434/LConn2
  L_168096434/LConn3 -- T_168096434_110000;33000;11000_Waipawa_substation/RConn3 -- bus159/LConn1
  T_367194918_110000;11000_Dannevirke_substation/RConn1 -- L_367194918/LConn1
  T_367194918_110000;11000_Dannevirke_substation/RConn2 -- L_367194918/LConn2
  L_367194918/LConn3 -- T_367194918_110000;11000_Dannevirke_substation/RConn3 -- bus160/LConn1
  T_180636348_110000;33000_Kensington_substation/RConn1 -- L_180636348/LConn1
  T_180636348_110000;33000_Kensington_substation/RConn2 -- L_180636348/LConn2
  L_180636348/LConn3 -- T_180636348_110000;33000_Kensington_substation/RConn3 -- bus161/LConn1
  T_101442986_110000;50000;33000_Maungatapere_substation/RConn1 -- L_101442986/LConn1
  T_101442986_110000;50000;33000_Maungatapere_substation/RConn2 -- L_101442986/LConn2
  L_101442986/LConn3 -- T_101442986_110000;50000;33000_Maungatapere_substation/RConn3 -- bus162/LConn1
  T_97334973_110000;33000_Mount_Maunganui_substation/RConn1 -- L_97334973/LConn1
  T_97334973_110000;33000_Mount_Maunganui_substation/RConn2 -- L_97334973/LConn2
  L_97334973/LConn3 -- T_97334973_110000;33000_Mount_Maunganui_substation/RConn3 -- bus163/LConn1
  T_160708893_110000;33000_Tauranga_substation/RConn1 -- L_160708893/LConn1
  T_160708893_110000;33000_Tauranga_substation/RConn2 -- L_160708893/LConn2
  L_160708893/LConn3 -- T_160708893_110000;33000_Tauranga_substation/RConn3 -- bus164/LConn1
  T_119877500_220000;110000;33000_Kaitimako_sub_station/RConn1 -- L_119877500/LConn1
  T_119877500_220000;110000;33000_Kaitimako_sub_station/RConn2 -- L_119877500/LConn2
  L_119877500/LConn3 -- T_119877500_220000;110000;33000_Kaitimako_sub_station/RConn3 -- bus165/LConn1
  T_410455856_110000;33000_Mangere_substation/RConn1 -- L_410455856/LConn1
  T_410455856_110000;33000_Mangere_substation/RConn2 -- L_410455856/LConn2
  L_410455856/LConn3 -- T_410455856_110000;33000_Mangere_substation/RConn3 -- bus166/LConn1
  T_269746976_110000;33000_Masterton_substation/RConn1 -- L_269746976/LConn1
  T_269746976_110000;33000_Masterton_substation/RConn2 -- L_269746976/LConn2
  L_269746976/LConn3 -- T_269746976_110000;33000_Masterton_substation/RConn3 -- bus167/LConn1
  T_167285978_110000;33000_Mangamaire_substation/RConn1 -- L_167285978/LConn1
  T_167285978_110000;33000_Mangamaire_substation/RConn2 -- L_167285978/LConn2
  L_167285978/LConn3 -- T_167285978_110000;33000_Mangamaire_substation/RConn3 -- bus168/LConn1
  T_25176792_110000;33000;11000_Central_Park_substation/RConn1 -- L_25176792/LConn1
  T_25176792_110000;33000;11000_Central_Park_substation/RConn2 -- L_25176792/LConn2
  L_25176792/LConn3 -- T_25176792_110000;33000;11000_Central_Park_substation/RConn3 -- bus169/LConn1
  T_95343089_220000;110000;33000_Wilton_substation/RConn1 -- L_95343089/LConn1
  T_95343089_220000;110000;33000_Wilton_substation/RConn2 -- L_95343089/LConn2
  L_95343089/LConn3 -- T_95343089_220000;110000;33000_Wilton_substation/RConn3 -- bus170/LConn1
  T_269748077_110000;11000_Woodville_substation/RConn1 -- L_269748077/LConn1
  T_269748077_110000;11000_Woodville_substation/RConn2 -- L_269748077/LConn2
  L_269748077/LConn3 -- T_269748077_110000;11000_Woodville_substation/RConn3 -- bus171/LConn1
  T_29545850_110000;33000;11000_Melling_substation/RConn1 -- L_29545850/LConn1
  T_29545850_110000;33000;11000_Melling_substation/RConn2 -- L_29545850/LConn2
  L_29545850/LConn3 -- T_29545850_110000;33000;11000_Melling_substation/RConn3 -- bus172/LConn1
  T_260242665_110000;22000_Kingsland_zone_substation/RConn1 -- L_260242665/LConn1
  T_260242665_110000;22000_Kingsland_zone_substation/RConn2 -- L_260242665/LConn2
  L_260242665/LConn3 -- T_260242665_110000;22000_Kingsland_zone_substation/RConn3 -- bus173/LConn1
  T_27030962_110000;22000_Mount_Roskill_substation/RConn1 -- L_27030962/LConn1
  T_27030962_110000;22000_Mount_Roskill_substation/RConn2 -- L_27030962/LConn2
  L_27030962/LConn3 -- T_27030962_110000;22000_Mount_Roskill_substation/RConn3 -- bus174/LConn1
  T_167952087_110000_Kaikohe_substation/RConn1 -- L_167952087/LConn1
  T_167952087_110000_Kaikohe_substation/RConn2 -- L_167952087/LConn2
  L_167952087/LConn3 -- T_167952087_110000_Kaikohe_substation/RConn3 -- bus175/LConn1
  T_352911643_110000;33000_Hineura_substation/RConn1 -- L_352911643/LConn1
  T_352911643_110000;33000_Hineura_substation/RConn2 -- L_352911643/LConn2
  L_352911643/LConn3 -- T_352911643_110000;33000_Hineura_substation/RConn3 -- bus176/LConn1
  T_161010976_110000;33000_Te_Matai_substation/RConn1 -- L_161010976/LConn1
  T_161010976_110000;33000_Te_Matai_substation/RConn2 -- L_161010976/LConn2
  L_161010976/LConn3 -- T_161010976_110000;33000_Te_Matai_substation/RConn3 -- bus177/LConn1
  T_154965833_110000;22000_Liverpool_zone_substation/RConn1 -- L_154965833/LConn1
  T_154965833_110000;22000_Liverpool_zone_substation/RConn2 -- L_154965833/LConn2
  L_154965833/LConn3 -- T_154965833_110000;22000_Liverpool_zone_substation/RConn3 -- bus178/LConn1
  T_87495237_110000_Penrose_substation_(110kV)/RConn1 -- L_87495237/LConn1
  T_87495237_110000_Penrose_substation_(110kV)/RConn2 -- L_87495237/LConn2
  L_87495237/LConn3 -- T_87495237_110000_Penrose_substation_(110kV)/RConn3 -- bus179/LConn1
  T_158810608_110000;22000;11000_Quay_zone_substation/RConn1 -- L_158810608/LConn1
  T_158810608_110000;22000;11000_Quay_zone_substation/RConn2 -- L_158810608/LConn2
  L_158810608/LConn3 -- T_158810608_110000;22000;11000_Quay_zone_substation/RConn3 -- bus180/LConn1
  T_272196494_110000;33000_Blenheim_substation/RConn1 -- L_272196494/LConn1
  T_272196494_110000;33000_Blenheim_substation/RConn2 -- L_272196494/LConn2
  L_272196494/LConn3 -- T_272196494_110000;33000_Blenheim_substation/RConn3 -- bus181/LConn1
  T_167705537_220000;110000;66000;33000_Stoke_substation/RConn1 -- L_167705537/LConn1
  T_167705537_220000;110000;66000;33000_Stoke_substation/RConn2 -- L_167705537/LConn2
  L_167705537/LConn3 -- T_167705537_220000;110000;66000;33000_Stoke_substation/RConn3 -- bus182/LConn1
  T_182456667_110000_/RConn1 -- L_182456667/LConn1
  T_182456667_110000_/RConn2 -- L_182456667/LConn2
  L_182456667/LConn3 -- T_182456667_110000_/RConn3 -- bus183/LConn1
  T_182466629__/RConn1 -- L_182466629/LConn1
  T_182466629__/RConn2 -- L_182466629/LConn2
  L_182466629/LConn3 -- T_182466629__/RConn3 -- bus184/LConn1
  T_269748078_110000_Te_Apiti_substation/RConn1 -- L_269748078/LConn1
  T_269748078_110000_Te_Apiti_substation/RConn2 -- L_269748078/LConn2
  L_269748078/LConn3 -- T_269748078_110000_Te_Apiti_substation/RConn3 -- bus185/LConn1
  T_93707134__/RConn1 -- L_93707134/LConn1
  T_93707134__/RConn2 -- L_93707134/LConn2
  L_93707134/LConn3 -- T_93707134__/RConn3 -- bus186/LConn1
  T_363290611__/RConn1 -- L_363290611/LConn1
  T_363290611__/RConn2 -- L_363290611/LConn2
  L_363290611/LConn3 -- T_363290611__/RConn3 -- bus187/LConn1
  T_95343088_110000;33000_Takapu_Road_substation/RConn1 -- L_95343088/LConn1
  T_95343088_110000;33000_Takapu_Road_substation/RConn2 -- L_95343088/LConn2
  L_95343088/LConn3 -- T_95343088_110000;33000_Takapu_Road_substation/RConn3 -- bus188/LConn1
  T_34937276_110000;33000_Pauatahanui_substation/RConn1 -- L_34937276/LConn1
  T_34937276_110000;33000_Pauatahanui_substation/RConn2 -- L_34937276/LConn2
  L_34937276/LConn3 -- T_34937276_110000;33000_Pauatahanui_substation/RConn3 -- bus189/LConn1
  T_193039355_110000_Mangaturoto_substation/RConn1 -- L_193039355/LConn1
  T_193039355_110000_Mangaturoto_substation/RConn2 -- L_193039355/LConn2
  L_193039355/LConn3 -- T_193039355_110000_Mangaturoto_substation/RConn3 -- bus190/LConn1
  T_100957314_220000;66000_Bromley_substation/RConn1 -- L_100957314/LConn1
  T_100957314_220000;66000_Bromley_substation/RConn2 -- L_100957314/LConn2
  L_100957314/LConn3 -- T_100957314_220000;66000_Bromley_substation/RConn3 -- bus191/LConn1
  T_33795353_220000;66000;33000_Islington_substation/RConn1 -- L_33795353/LConn1
  T_33795353_220000;66000;33000_Islington_substation/RConn2 -- L_33795353/LConn2
  L_33795353/LConn3 -- T_33795353_220000;66000;33000_Islington_substation/RConn3 -- bus192/LConn1
  T_268826084_220000;66000;33000_Ashburton_substation/RConn1 -- L_268826084/LConn1
  T_268826084_220000;66000;33000_Ashburton_substation/RConn2 -- L_268826084/LConn2
  L_268826084/LConn3 -- T_268826084_220000;66000;33000_Ashburton_substation/RConn3 -- bus193/LConn1
  T_329266069__/RConn1 -- L_329266069/LConn1
  T_329266069__/RConn2 -- L_329266069/LConn2
  L_329266069/LConn3 -- T_329266069__/RConn3 -- bus194/LConn1
  T_180514007_220000;110000_Roxburgh_substation/RConn1 -- L_180514007/LConn1
  T_180514007_220000;110000_Roxburgh_substation/RConn2 -- L_180514007/LConn2
  L_180514007/LConn3 -- T_180514007_220000;110000_Roxburgh_substation/RConn3 -- bus195/LConn1
  T_414953388_220000;33000_Naesby_substation/RConn1 -- L_414953388/LConn1
  T_414953388_220000;33000_Naesby_substation/RConn2 -- L_414953388/LConn2
  L_414953388/LConn3 -- T_414953388_220000;33000_Naesby_substation/RConn3 -- bus196/LConn1
  T_232382576_220000;110000_Marsden_substation/RConn1 -- L_232382576/LConn1
  T_232382576_220000;110000_Marsden_substation/RConn2 -- L_232382576/LConn2
  L_232382576/LConn3 -- T_232382576_220000;110000_Marsden_substation/RConn3 -- bus197/LConn1
  T_270556206_220000_Ohaaki_substation/RConn1 -- L_270556206/LConn1
  T_270556206_220000_Ohaaki_substation/RConn2 -- L_270556206/LConn2
  L_270556206/LConn3 -- T_270556206_220000_Ohaaki_substation/RConn3 -- bus198/LConn1
  T_329266072__/RConn1 -- L_329266072/LConn1
  T_329266072__/RConn2 -- L_329266072/LConn2
  L_329266072/LConn3 -- T_329266072__/RConn3 -- bus199/LConn1
  T_270018358_220000_Aratiatia_substation/RConn1 -- L_270018358/LConn1
  T_270018358_220000_Aratiatia_substation/RConn2 -- L_270018358/LConn2
  L_270018358/LConn3 -- T_270018358_220000_Aratiatia_substation/RConn3 -- bus200/LConn1
  T_255873374_220000_Ngatamariki_substation/RConn1 -- L_255873374/LConn1
  T_255873374_220000_Ngatamariki_substation/RConn2 -- L_255873374/LConn2
  L_255873374/LConn3 -- T_255873374_220000_Ngatamariki_substation/RConn3 -- bus201/LConn1
  T_270554679_220000_Nga_Awa_Purua_substation/RConn1 -- L_270554679/LConn1
  T_270554679_220000_Nga_Awa_Purua_substation/RConn2 -- L_270554679/LConn2
  L_270554679/LConn3 -- T_270554679_220000_Nga_Awa_Purua_substation/RConn3 -- bus202/LConn1
  T_89664063_220000_Benmore_(HVAC)_substation/RConn1 -- L_89664063/LConn1
  T_89664063_220000_Benmore_(HVAC)_substation/RConn2 -- L_89664063/LConn2
  L_89664063/LConn3 -- T_89664063_220000_Benmore_(HVAC)_substation/RConn3 -- bus203/LConn1
  T_94840399_220000_Livingstone_switching_station/RConn1 -- L_94840399/LConn1
  T_94840399_220000_Livingstone_switching_station/RConn2 -- L_94840399/LConn2
  L_94840399/LConn3 -- T_94840399_220000_Livingstone_switching_station/RConn3 -- bus204/LConn1
  T_89636510_220000_Ohau_A_substation/RConn1 -- L_89636510/LConn1
  T_89636510_220000_Ohau_A_substation/RConn2 -- L_89636510/LConn2
  L_89636510/LConn3 -- T_89636510_220000_Ohau_A_substation/RConn3 -- bus205/LConn1
  T_170300247_220000;33000_Twizel_substation/RConn1 -- L_170300247/LConn1
  T_170300247_220000;33000_Twizel_substation/RConn2 -- L_170300247/LConn2
  L_170300247/LConn3 -- T_170300247_220000;33000_Twizel_substation/RConn3 -- bus206/LConn1
  T_89636266_220000_Ohau_C_substation/RConn1 -- L_89636266/LConn1
  T_89636266_220000_Ohau_C_substation/RConn2 -- L_89636266/LConn2
  L_89636266/LConn3 -- T_89636266_220000_Ohau_C_substation/RConn3 -- bus207/LConn1
  T_89411122_220000;33000_Tokaanu_substation/RConn1 -- L_89411122/LConn1
  T_89411122_220000;33000_Tokaanu_substation/RConn2 -- L_89411122/LConn2
  L_89411122/LConn3 -- T_89411122_220000;33000_Tokaanu_substation/RConn3 -- bus208/LConn1
  T_87837416_220000_Whakamaru_substation/RConn1 -- L_87837416/LConn1
  T_87837416_220000_Whakamaru_substation/RConn2 -- L_87837416/LConn2
  L_87837416/LConn3 -- T_87837416_220000_Whakamaru_substation/RConn3 -- bus209/LConn1
  T_89637173_220000;110000;33000;11000_Waitaki_substation/RConn1 -- L_89637173/LConn1
  T_89637173_220000;110000;33000;11000_Waitaki_substation/RConn2 -- L_89637173/LConn2
  L_89637173/LConn3 -- T_89637173_220000;110000;33000;11000_Waitaki_substation/RConn3 -- bus210/LConn1
  T_89637174_220000_Aviemore_substation/RConn1 -- L_89637174/LConn1
  T_89637174_220000_Aviemore_substation/RConn2 -- L_89637174/LConn2
  L_89637174/LConn3 -- T_89637174_220000_Aviemore_substation/RConn3 -- bus211/LConn1
  T_89664057_350000;220000_Benmore_HVDC_static_inverter_station/RConn1 -- L_89664057/LConn1
  T_89664057_350000;220000_Benmore_HVDC_static_inverter_station/RConn2 -- L_89664057/LConn2
  L_89664057/LConn3 -- T_89664057_350000;220000_Benmore_HVDC_static_inverter_station/RConn3 -- bus212/LConn1
  T_89635947_220000_Ohau_B_substation/RConn1 -- L_89635947/LConn1
  T_89635947_220000_Ohau_B_substation/RConn2 -- L_89635947/LConn2
  L_89635947/LConn3 -- T_89635947_220000_Ohau_B_substation/RConn3 -- bus213/LConn1
  T_270550888__Maraetai_I_substation/RConn1 -- L_270550888/LConn1
  T_270550888__Maraetai_I_substation/RConn2 -- L_270550888/LConn2
  L_270550888/LConn3 -- T_270550888__Maraetai_I_substation/RConn3 -- bus214/LConn1
  T_167285260_220000;33000_Wairakei_substation/RConn1 -- L_167285260/LConn1
  T_167285260_220000;33000_Wairakei_substation/RConn2 -- L_167285260/LConn2
  L_167285260/LConn3 -- T_167285260_220000;33000_Wairakei_substation/RConn3 -- bus215/LConn1
  T_412588974_220000_Tiwai_substation/RConn1 -- L_412588974/LConn1
  T_412588974_220000_Tiwai_substation/RConn2 -- L_412588974/LConn2
  L_412588974/LConn3 -- T_412588974_220000_Tiwai_substation/RConn3 -- bus216/LConn1
  T_268841395_220000_North_Makarewa_substation/RConn1 -- L_268841395/LConn1
  T_268841395_220000_North_Makarewa_substation/RConn2 -- L_268841395/LConn2
  L_268841395/LConn3 -- T_268841395_220000_North_Makarewa_substation/RConn3 -- bus217/LConn1
  T_87897292_220000_Southdown_substation/RConn1 -- L_87897292/LConn1
  T_87897292_220000_Southdown_substation/RConn2 -- L_87897292/LConn2
  L_87897292/LConn3 -- T_87897292_220000_Southdown_substation/RConn3 -- bus218/LConn1
  T_169512273__/RConn1 -- L_169512273/LConn1
  T_169512273__/RConn2 -- L_169512273/LConn2
  L_169512273/LConn3 -- T_169512273__/RConn3 -- bus219/LConn1
  T_87928925__Maraetai_II_sub_station/RConn1 -- L_87928925/LConn1
  T_87928925__Maraetai_II_sub_station/RConn2 -- L_87928925/LConn2
  L_87928925/LConn3 -- T_87928925__Maraetai_II_sub_station/RConn3 -- bus220/LConn1
  T_341099346__Pakuranga_substation_(new)/RConn1 -- L_341099346/LConn1
  T_341099346__Pakuranga_substation_(new)/RConn2 -- L_341099346/LConn2
  L_341099346/LConn3 -- T_341099346__Pakuranga_substation_(new)/RConn3 -- bus221/LConn1
  T_156094589_220000_Brownhill_substation/RConn1 -- L_156094589/LConn1
  T_156094589_220000_Brownhill_substation/RConn2 -- L_156094589/LConn2
  L_156094589/LConn3 -- T_156094589_220000_Brownhill_substation/RConn3 -- bus222/LConn1
  T_167283894_220000;110000;33000_Edgecumbe_substation/RConn1 -- L_167283894/LConn1
  T_167283894_220000;110000;33000_Edgecumbe_substation/RConn2 -- L_167283894/LConn2
  L_167283894/LConn3 -- T_167283894_220000;110000;33000_Edgecumbe_substation/RConn3 -- bus223/LConn1
  T_93713118_220000;110000;33000;11000_Haywards_substation/RConn1 -- L_93713118/LConn1
  T_93713118_220000;110000;33000;11000_Haywards_substation/RConn2 -- L_93713118/LConn2
  L_93713118/LConn3 -- T_93713118_220000;110000;33000;11000_Haywards_substation/RConn3 -- bus224/LConn1
  T_272522517_220000_Ohakuri_substation/RConn1 -- L_272522517/LConn1
  T_272522517_220000_Ohakuri_substation/RConn2 -- L_272522517/LConn2
  L_272522517/LConn3 -- T_272522517_220000_Ohakuri_substation/RConn3 -- bus225/LConn1
  T_270012796_220000_Tekapo_B_substation/RConn1 -- L_270012796/LConn1
  T_270012796_220000_Tekapo_B_substation/RConn2 -- L_270012796/LConn2
  L_270012796/LConn3 -- T_270012796_220000_Tekapo_B_substation/RConn3 -- bus226/LConn1
  T_412589726_220000_Manapouri_substation/RConn1 -- L_412589726/LConn1
  T_412589726_220000_Manapouri_substation/RConn2 -- L_412589726/LConn2
  L_412589726/LConn3 -- T_412589726_220000_Manapouri_substation/RConn3 -- bus227/LConn1
